simulink model "ElevatorPlant_Storage_A"  (R2015b)
(part 6 of 8)

              BUT_1=BUT_TEMP;
              FIRST_BUT=false;
            state Button_CAR_2
              en:
              BUTTON_CAR(3)=true;
              BUT_TEMP=2;
              LPC2=true;
              PUSHED=true;
              UPDATE=false;
              IN_LL=false; ET_LL=0;
            state First_but_2
              en:
              BUT_1=BUT_TEMP;
              FIRST_BUT=false;
            state Button_CAR_3
              en:
              BUTTON_CAR(4)=true;
              BUT_TEMP=3;
              LPC3=true;
              PUSHED=true;
              UPDATE=false;
              IN_LL=false; ET_LL=0;
            state First_but_3
              en:
              BUT_1=BUT_TEMP;
              FIRST_BUT=false;
            (default) -> (junction 91635)
            (junction 91635) -> Emergency.Doors.Opening0.Button_detection.BUTTON_CAR.Button_CAR_0 [order 1] : [P0]
            Emergency.Doors.Opening0.Button_detection.BUTTON_CAR.Button_CAR_0 -> (junction 91636)
            (junction 91636) -> Emergency.Doors.Opening0.Button_detection.BUTTON_CAR.First_but_0 [order 1] : [FIRST_BUT && not(RPC0)]
            Emergency.Doors.Opening0.Button_detection.BUTTON_CAR.First_but_0 -> (junction 91637)
            (junction 91635) -> (junction 91638) [order 2]
            (junction 91636) -> (junction 91639) [order 2]
            (junction 91637) -> (junction 91640)
            (junction 91639) -> (junction 91638)
            (junction 91640) -> (junction 91639)
            (junction 91638) -> (junction 91643)
            Emergency.Doors.Opening0.Button_detection.BUTTON_CAR.Button_CAR_1 -> (junction 91641)
            (junction 91641) -> Emergency.Doors.Opening0.Button_detection.BUTTON_CAR.First_but_1 [order 1] : [FIRST_BUT && not(RPC1)]
            Emergency.Doors.Opening0.Button_detection.BUTTON_CAR.First_but_1 -> (junction 91642)
            (junction 91641) -> (junction 91645) [order 2]
            (junction 91642) -> (junction 91646)
            (junction 91643) -> Emergency.Doors.Opening0.Button_detection.BUTTON_CAR.Button_CAR_1 [order 1] : [P1]
            (junction 91643) -> (junction 91644) [order 2]
            (junction 91645) -> (junction 91644)
            (junction 91646) -> (junction 91645)
            (junction 91644) -> (junction 91647)
            (junction 91647) -> Emergency.Doors.Opening0.Button_detection.BUTTON_CAR.Button_CAR_2 [order 1] : [P2]
            Emergency.Doors.Opening0.Button_detection.BUTTON_CAR.Button_CAR_2 -> (junction 91648)
            (junction 91648) -> Emergency.Doors.Opening0.Button_detection.BUTTON_CAR.First_but_2 [order 1] : [FIRST_BUT && not(RPC2)]
            Emergency.Doors.Opening0.Button_detection.BUTTON_CAR.First_but_2 -> (junction 91649)
            (junction 91647) -> (junction 91650) [order 2]
            (junction 91648) -> (junction 91651) [order 2]
            (junction 91649) -> (junction 91652)
            (junction 91651) -> (junction 91650)
            (junction 91652) -> (junction 91651)
            (junction 91650) -> (junction 91653)
            (junction 91653) -> Emergency.Doors.Opening0.Button_detection.BUTTON_CAR.Button_CAR_3 [order 1] : [P3]
            Emergency.Doors.Opening0.Button_detection.BUTTON_CAR.Button_CAR_3 -> (junction 91654)
            (junction 91654) -> Emergency.Doors.Opening0.Button_detection.BUTTON_CAR.First_but_3 [order 1] : [FIRST_BUT && not(RPC3)]
            Emergency.Doors.Opening0.Button_detection.BUTTON_CAR.First_but_3 -> (junction 91655)
            (junction 91653) -> (junction 91656) [order 2]
            (junction 91654) -> (junction 91657) [order 2]
            (junction 91655) -> (junction 91658)
            (junction 91657) -> (junction 91656)
            (junction 91658) -> (junction 91657)
          state BUTTON_UP
            state Button_UP_0
              en:
              BUTTON_UP(1)=true;
              BUT_TEMP=0;
              LPS0=true;
              PUSHED=true;
              UPDATE=false;
              IN_LL=false; ET_LL=0;
            state First_but_0
              en:
              BUT_1=BUT_TEMP;
              FIRST_BUT=false;
            state Button_UP_1
              en:
              BUTTON_UP(2)=true;
              BUT_TEMP=1;
              LPS1=true;
              PUSHED=true;
              UPDATE=false;
              IN_LL=false; ET_LL=0;
            state First_but_1
              en:
              BUT_1=BUT_TEMP;
              FIRST_BUT=false;
            state Button_UP_2
              en:
              BUTTON_UP(3)=true;
              BUT_TEMP=2;
              LPS2=true;
              PUSHED=true;
              UPDATE=false;
              IN_LL=false; ET_LL=0;
            state First_but_2
              en:
              BUT_1=BUT_TEMP;
              FIRST_BUT=false;
            (junction 91708) -> Emergency.Doors.Opening0.Button_detection.BUTTON_UP.Button_UP_0 [order 1] : [PS0]
            Emergency.Doors.Opening0.Button_detection.BUTTON_UP.Button_UP_0 -> (junction 91709)
            (junction 91709) -> Emergency.Doors.Opening0.Button_detection.BUTTON_UP.First_but_0 [order 1] : [FIRST_BUT && not(RPC0)]
            Emergency.Doors.Opening0.Button_detection.BUTTON_UP.First_but_0 -> (junction 91710)
            (default) -> (junction 91708)
            (junction 91708) -> (junction 91713) [order 2]
            (junction 91709) -> (junction 91711) [order 2]
            (junction 91710) -> (junction 91712)
            (junction 91712) -> (junction 91711)
            (junction 91711) -> (junction 91713)
            (junction 91713) -> (junction 91714)
            (junction 91714) -> Emergency.Doors.Opening0.Button_detection.BUTTON_UP.Button_UP_1 [order 1] : [PS1]
            Emergency.Doors.Opening0.Button_detection.BUTTON_UP.Button_UP_1 -> (junction 91715)
            (junction 91715) -> Emergency.Doors.Opening0.Button_detection.BUTTON_UP.First_but_1 [order 1] : [FIRST_BUT && not(RPC1)]
            Emergency.Doors.Opening0.Button_detection.BUTTON_UP.First_but_1 -> (junction 91716)
            (junction 91714) -> (junction 91717) [order 2]
            (junction 91715) -> (junction 91718) [order 2]
            (junction 91716) -> (junction 91719)
            (junction 91718) -> (junction 91717)
            (junction 91719) -> (junction 91718)
            (junction 91717) -> (junction 91721)
            Emergency.Doors.Opening0.Button_detection.BUTTON_UP.First_but_2 -> (junction 91720)
            (junction 91720) -> (junction 91725)
            (junction 91721) -> Emergency.Doors.Opening0.Button_detection.BUTTON_UP.Button_UP_2 [order 1] : [PS2]
            Emergency.Doors.Opening0.Button_detection.BUTTON_UP.Button_UP_2 -> (junction 91722)
            (junction 91722) -> Emergency.Doors.Opening0.Button_detection.BUTTON_UP.First_but_2 [order 1] : [FIRST_BUT && not(RPC2)]
            (junction 91721) -> (junction 91723) [order 2]
            (junction 91722) -> (junction 91724) [order 2]
            (junction 91724) -> (junction 91723)
            (junction 91725) -> (junction 91724)
          state Max_Min_assignment
            state Min_but
              en:
              BUTTON=MIN_BUT;
            state Max_but
              en:
              BUTTON=MAX_BUT;
            state First_but
              en:
              BUTTON=BUT_1;
            state Max_but1
              en:
              MAX_BUT=2;
            state Max_but2
              en:
              MAX_BUT=1;
            state Max_but3
              en:
              MAX_BUT=0;
            state Min_but1
              en:
              MIN_BUT=1;
            state Min_but2
              en:
              MIN_BUT=2;
            state Min_but3
              en:
              MIN_BUT=3;
            state MAX
              en:
              MAX_BUT=BUT_TEMP;
            state MIN
              en:
              MIN_BUT=BUT_TEMP;
            state Updating_button_0
              en:
              BUTTON=MAX_BUT;
            state Updating_button_1
              en:
              BUTTON=MIN_BUT;
            (junction 91763) -> Emergency.Doors.Opening0.Button_detection.Max_Min_assignment.Min_but [order 1] : [(MAX_BUT-FLOOR)>(FLOOR-MIN_BUT)]
            Emergency.Doors.Opening0.Button_detection.Max_Min_assignment.Min_but -> (junction 91764)
            (junction 91765) -> (junction 91763) [order 1] : [not(FLAG_STOP) && MOTION==2 && FLAG==3]
            (default) -> (junction 91765)
            (junction 91763) -> (junction 91766) [order 2]
            (junction 91764) -> (junction 91767)
            (junction 91765) -> (junction 91768) [order 2]
            (junction 91766) -> Emergency.Doors.Opening0.Button_detection.Max_Min_assignment.Max_but [order 1] : [(MAX_BUT-FLOOR)<(FLOOR-MIN_BUT)]
            Emergency.Doors.Opening0.Button_detection.Max_Min_assignment.Max_but -> (junction 91767)
            (junction 91766) -> Emergency.Doors.Opening0.Button_detection.Max_Min_assignment.First_but [order 2]
            (junction 91767) -> (junction 91770)
            Emergency.Doors.Opening0.Button_detection.Max_Min_assignment.First_but -> (junction 91769)
            (junction 91769) -> (junction 91768)
            (junction 91770) -> (junction 91769)
            (junction 91768) -> (junction 91771)
            (junction 91772) -> (junction 91773) [order 1] : [MOTION==0]
                | {MOTION=1;
                | UPDATE=true;}
            (junction 91773) -> Emergency.Doors.Opening0.Button_detection.Max_Min_assignment.Max_but1 [order 1] : [BUTTON_UP(2)]
            Emergency.Doors.Opening0.Button_detection.Max_Min_assignment.Max_but1 -> (junction 91774)
            (junction 91771) -> (junction 91772) [order 1] : [BUTTON==FLOOR && EXTEND]
                | {EXTEND=false;}
            (junction 91771) -> (junction 91785) [order 2]
            (junction 91772) -> (junction 91777) [order 2]
            (junction 91773) -> (junction 91775) [order 2]
            (junction 91774) -> (junction 91776)
            (junction 91775) -> Emergency.Doors.Opening0.Button_detection.Max_Min_assignment.Max_but2 [order 1] : [BUTTON_UP(1)]
            Emergency.Doors.Opening0.Button_detection.Max_Min_assignment.Max_but2 -> (junction 91776)
            (junction 91775) -> Emergency.Doors.Opening0.Button_detection.Max_Min_assignment.Max_but3 [order 2]
            (junction 91776) -> (junction 91779)
            Emergency.Doors.Opening0.Button_detection.Max_Min_assignment.Max_but3 -> (junction 91778)
            (junction 91778) -> (junction 91777)
            (junction 91779) -> (junction 91778)
            (junction 91777) -> (junction 91780)
            (junction 91780) -> (junction 91781) [order 1] : [MOTION==1]
                | {MOTION=0;
                | UPDATE=true;}
            (junction 91781) -> Emergency.Doors.Opening0.Button_detection.Max_Min_assignment.Min_but1 [order 1] : [BUTTON_DOWN(1)]
            Emergency.Doors.Opening0.Button_detection.Max_Min_assignment.Min_but1 -> (junction 91782)
            (junction 91780) -> (junction 91786) [order 2]
            (junction 91781) -> (junction 91783) [order 2]
            (junction 91782) -> (junction 91784)
            (junction 91783) -> Emergency.Doors.Opening0.Button_detection.Max_Min_assignment.Min_but2 [order 1] : [BUTTON_DOWN(2)]
            Emergency.Doors.Opening0.Button_detection.Max_Min_assignment.Min_but2 -> (junction 91784)
            (junction 91783) -> Emergency.Doors.Opening0.Button_detection.Max_Min_assignment.Min_but3 [order 2]
            (junction 91784) -> (junction 91788)
            Emergency.Doors.Opening0.Button_detection.Max_Min_assignment.Min_but3 -> (junction 91787)
            (junction 91786) -> (junction 91785)
            (junction 91787) -> (junction 91786)
            (junction 91788) -> (junction 91787)
            (junction 91785) -> (junction 91790)
            Emergency.Doors.Opening0.Button_detection.Max_Min_assignment.MAX -> (junction 91789)
            (junction 91790) -> (junction 91791) [order 1] : [PUSHED]
            (junction 91791) -> (junction 91792) [order 1] : [not(BUT_TEMP==FLOOR) || not(MOTION==2)]
            (junction 91792) -> Emergency.Doors.Opening0.Button_detection.Max_Min_assignment.MAX [order 1] : [MAX_BUT<BUT_TEMP && not(UPDATE)]
            (junction 91789) -> (junction 91794)
            (junction 91790) -> (junction 91804) [order 2]
            (junction 91791) -> (junction 91797) [order 2]
            (junction 91792) -> (junction 91793) [order 2]
            (junction 91794) -> (junction 91793)
            (junction 91793) -> (junction 91795)
            (junction 91795) -> Emergency.Doors.Opening0.Button_detection.Max_Min_assignment.MIN [order 1] : [MIN_BUT>BUT_TEMP && not(UPDATE)]
            Emergency.Doors.Opening0.Button_detection.Max_Min_assignment.MIN -> (junction 91796)
            (junction 91795) -> (junction 91798) [order 2]
            (junction 91796) -> (junction 91799)
            (junction 91798) -> (junction 91797)
            (junction 91799) -> (junction 91798)
            (junction 91797) -> (junction 91800)
            (junction 91800) -> Emergency.Doors.Opening0.Button_detection.Max_Min_assignment.Updating_button_0 [order 1] : [MOTION==0]
            Emergency.Doors.Opening0.Button_detection.Max_Min_assignment.Updating_button_0 -> (junction 91801)
            (junction 91800) -> (junction 91802) [order 2]
            (junction 91801) -> (junction 91803)
            (junction 91802) -> Emergency.Doors.Opening0.Button_detection.Max_Min_assignment.Updating_button_1 [order 1] : [MOTION==1]
            Emergency.Doors.Opening0.Button_detection.Max_Min_assignment.Updating_button_1 -> (junction 91803)
            (junction 91802) -> (junction 91805) [order 2]
            (junction 91803) -> (junction 91806)
            (junction 91805) -> (junction 91804)
            (junction 91806) -> (junction 91805)
          state GoTo_PositionControl
            en:
            BUTTON=BUT_TEMP;
            FLAG=2;
          state Emergency
            en:
            FLAG_EMG=true;
            FLAG=4;
          state Timer_EME
            state Set_tmr
              en:
              Q_EME=true;
            state Counting
              en:
              ET_EME= ET_EME + 1;
              Q_EME=false;
            state Set
              en:
              IN_EME=true;
              PT_EME=3;
            (junction 91896) -> Emergency.Doors.Opening0.Button_detection.Timer_EME.Set_tmr [order 1] : [ET_EME==PT_EME]
            Emergency.Doors.Opening0.Button_detection.Timer_EME.Set_tmr -> (junction 91897)
            Emergency.Doors.Opening0.Button_detection.Timer_EME.Counting -> (junction 91896)
            (junction 91896) -> (junction 91897) [order 2]
            (default) -> Emergency.Doors.Opening0.Button_detection.Timer_EME.Set
            Emergency.Doors.Opening0.Button_detection.Timer_EME.Set -> (junction 91898)
            (junction 91898) -> Emergency.Doors.Opening0.Button_detection.Timer_EME.Counting [order 1] : [ET_EME<PT_EME]
            (junction 91898) -> (junction 91897) [order 2]
          state Not_Emergency
            en:
            IN_EME=false;
            ET_EME=0;
          state SwitchingOFF_LEDs
            en:
            LPD3=false;
            LPD2=false;
            LPS2=false;
            LPD1=false;
            LPS1=false;
            LPS0=false;
          (default) -> (junction 91497)
          (junction 91497) -> (junction 91498) [order 1] : [FLAG==1 && not(PUSHED)]
              | {BUTTON=FLOOR;
              | BUT_TEMP=BUTTON;
              | BUT_1=FLOOR;}
          (junction 91498) -> Emergency.Doors.Opening0.Button_detection.Timer_LL [order 1] : [not(FLAG_STOP)]
          Emergency.Doors.Opening0.Button_detection.Timer_LL -> Emergency.Doors.Opening0.Button_detection.Save_energy
          Emergency.Doors.Opening0.Button_detection.Save_energy -> (junction 91499)
          (junction 91497) -> (junction 91500) [order 2]
          (junction 91498) -> (junction 91501) [order 2]
          (junction 91499) -> (junction 91502)
          (junction 91501) -> (junction 91500)
          (junction 91502) -> (junction 91501)
          (junction 91500) -> Emergency.Doors.Opening0.Button_detection.BUTTON_CAR
          Emergency.Doors.Opening0.Button_detection.BUTTON_UP -> Emergency.Doors.Opening0.Button_detection.BUTTON_DOWN
          Emergency.Doors.Opening0.Button_detection.BUTTON_DOWN -> Emergency.Doors.Opening0.Button_detection.Max_Min_assignment
          Emergency.Doors.Opening0.Button_detection.Max_Min_assignment -> (junction 91503)
          Emergency.Doors.Opening0.Button_detection.BUTTON_CAR -> Emergency.Doors.Opening0.Button_detection.BUTTON_UP
          (junction 91503) -> (junction 91505)
          (junction 91505) -> (junction 91504)
          (junction 91504) -> (junction 91506)
          (junction 91506) -> (junction 91507) [order 1] : [FLAG==1]
          (junction 91507) -> Emergency.Doors.Opening0.Button_detection.GoTo_PositionControl [order 1] : [PUSHED]
          Emergency.Doors.Opening0.Button_detection.GoTo_PositionControl -> (junction 91508)
          (junction 91506) -> (junction 91518) [order 2]
          (junction 91507) -> (junction 91509) [order 2]
          (junction 91508) -> (junction 91510)
          (junction 91510) -> (junction 91509)
          (junction 91509) -> (junction 91512)
          Emergency.Doors.Opening0.Button_detection.Emergency -> (junction 91511)
          (junction 91512) -> Emergency.Doors.Opening0.Button_detection.Timer_EME [order 1] : [STOP]
              | {IN_LL=false; ET_LL=0;FLAG=1;}
          Emergency.Doors.Opening0.Button_detection.Timer_EME -> (junction 91513)
          (junction 91513) -> Emergency.Doors.Opening0.Button_detection.Emergency [order 1] : [Q_EME]
          (junction 91511) -> (junction 91515)
          (junction 91512) -> Emergency.Doors.Opening0.Button_detection.Not_Emergency [order 2]
          (junction 91513) -> (junction 91514) [order 2]
          (junction 91515) -> (junction 91514)
          (junction 91514) -> (junction 91517)
          Emergency.Doors.Opening0.Button_detection.Not_Emergency -> (junction 91517)
          Emergency.Doors.Opening0.Button_detection.SwitchingOFF_LEDs -> (junction 91516)
          (junction 91517) -> Emergency.Doors.Opening0.Button_detection.SwitchingOFF_LEDs [order 1] : [FLAG_STOP && FLAG==2]
          (junction 91516) -> (junction 91520)
          (junction 91517) -> (junction 91519) [order 2]
          (junction 91519) -> (junction 91518)
          (junction 91520) -> (junction 91519)
        state Button_detection1
          state Save_energy
            en:
            LL=not(Q_LL);
          state Timer_LL
            state Set_tmr
              en:
              Q_LL=true;
            state Counting
              en:
              ET_LL= ET_LL + 1;
              Q_LL=false;
            state Set
              en:
              IN_LL=true;
              PT_LL=10;
            (junction 91981) -> Emergency.Doors.Opening0.Button_detection1.Timer_LL.Set_tmr [order 1] : [ET_LL==PT_LL]
            Emergency.Doors.Opening0.Button_detection1.Timer_LL.Set_tmr -> (junction 91982)
            Emergency.Doors.Opening0.Button_detection1.Timer_LL.Counting -> (junction 91981)
            (junction 91981) -> (junction 91982) [order 2]
            (default) -> Emergency.Doors.Opening0.Button_detection1.Timer_LL.Set
            Emergency.Doors.Opening0.Button_detection1.Timer_LL.Set -> (junction 91983)
            (junction 91983) -> Emergency.Doors.Opening0.Button_detection1.Timer_LL.Counting [order 1] : [ET_LL<PT_LL]
            (junction 91983) -> (junction 91982) [order 2]
          state BUTTON_DOWN
            state Button_DOWN_1
              en:
              BUTTON_DOWN(2)=true;
              BUT_TEMP=1;
              LPD1=true;
              PUSHED=true;
              UPDATE=false;
              IN_LL=false; ET_LL=0;
            state First_but_1
              en:
              BUT_1=BUT_TEMP;
              FIRST_BUT=false;
            state Button_DOWN_2
              en:
              BUTTON_DOWN(3)=true;
              BUT_TEMP=2;
              LPD2=true;
              PUSHED=true;
              UPDATE=false;
              IN_LL=false; ET_LL=0;
            state First_but_2
              en:
              BUT_1=BUT_TEMP;
              FIRST_BUT=false;
            state Button_DOWN_3
              en:
              BUTTON_DOWN(4)=true;
              BUT_TEMP=3;
              LPD3=true;
              PUSHED=true;
              UPDATE=false;
              IN_LL=false; ET_LL=0;
            state First_but_3
              en:
              BUT_1=BUT_TEMP;
              FIRST_BUT=false;
            (default) -> (junction 91996)
            (junction 91996) -> Emergency.Doors.Opening0.Button_detection1.BUTTON_DOWN.Button_DOWN_1 [order 1] : [PD1]
            Emergency.Doors.Opening0.Button_detection1.BUTTON_DOWN.Button_DOWN_1 -> (junction 91997)
            (junction 91997) -> Emergency.Doors.Opening0.Button_detection1.BUTTON_DOWN.First_but_1 [order 1] : [FIRST_BUT && not(RPC1)]
            Emergency.Doors.Opening0.Button_detection1.BUTTON_DOWN.First_but_1 -> (junction 91998)
            (junction 91996) -> (junction 91999) [order 2]
            (junction 91997) -> (junction 92000) [order 2]
            (junction 91998) -> (junction 92001)
            (junction 92000) -> (junction 91999)
            (junction 92001) -> (junction 92000)
            (junction 91999) -> (junction 92002)
            (junction 92002) -> Emergency.Doors.Opening0.Button_detection1.BUTTON_DOWN.Button_DOWN_2 [order 1] : [PD2]
            Emergency.Doors.Opening0.Button_detection1.BUTTON_DOWN.Button_DOWN_2 -> (junction 92003)
            (junction 92003) -> Emergency.Doors.Opening0.Button_detection1.BUTTON_DOWN.First_but_2 [order 1] : [FIRST_BUT && not(RPC2)]
            Emergency.Doors.Opening0.Button_detection1.BUTTON_DOWN.First_but_2 -> (junction 92004)
            (junction 92002) -> (junction 92005) [order 2]
            (junction 92003) -> (junction 92006) [order 2]
            (junction 92004) -> (junction 92007)
            (junction 92006) -> (junction 92005)
            (junction 92007) -> (junction 92006)
            (junction 92005) -> (junction 92008)
            (junction 92008) -> Emergency.Doors.Opening0.Button_detection1.BUTTON_DOWN.Button_DOWN_3 [order 1] : [PD3]
            Emergency.Doors.Opening0.Button_detection1.BUTTON_DOWN.Button_DOWN_3 -> (junction 92009)
            (junction 92009) -> Emergency.Doors.Opening0.Button_detection1.BUTTON_DOWN.First_but_3 [order 1] : [FIRST_BUT && not(RPC3)]
            Emergency.Doors.Opening0.Button_detection1.BUTTON_DOWN.First_but_3 -> (junction 92010)
            (junction 92008) -> (junction 92011) [order 2]
            (junction 92009) -> (junction 92012) [order 2]
            (junction 92010) -> (junction 92013)
            (junction 92012) -> (junction 92011)
            (junction 92013) -> (junction 92012)
          state BUTTON_CAR
            state Button_CAR_0
              en:
              BUTTON_CAR(1)=true;
              BUT_TEMP=0;
              LPC0=true;
              PUSHED=true;
              UPDATE=false;
              IN_LL=false; ET_LL=0;
            state First_but_0
              en:
              BUT_1=BUT_TEMP;
              FIRST_BUT=false;
            state Button_CAR_1
              en:
              BUTTON_CAR(2)=true;
              BUT_TEMP=1;
              LPC1=true;
              PUSHED=true;
              UPDATE=false;
              IN_LL=false; ET_LL=0;
            state First_but_1
              en:
              BUT_1=BUT_TEMP;
              FIRST_BUT=false;
            state Button_CAR_2
              en:
              BUTTON_CAR(3)=true;
              BUT_TEMP=2;
              LPC2=true;
              PUSHED=true;
              UPDATE=false;
              IN_LL=false; ET_LL=0;
            state First_but_2
              en:
              BUT_1=BUT_TEMP;
              FIRST_BUT=false;
            state Button_CAR_3
              en:
              BUTTON_CAR(4)=true;
              BUT_TEMP=3;
              LPC3=true;
              PUSHED=true;
              UPDATE=false;
              IN_LL=false; ET_LL=0;
            state First_but_3
              en:
              BUT_1=BUT_TEMP;
              FIRST_BUT=false;
            (default) -> (junction 92051)
            (junction 92051) -> Emergency.Doors.Opening0.Button_detection1.BUTTON_CAR.Button_CAR_0 [order 1] : [P0]
            Emergency.Doors.Opening0.Button_detection1.BUTTON_CAR.Button_CAR_0 -> (junction 92052)
            (junction 92052) -> Emergency.Doors.Opening0.Button_detection1.BUTTON_CAR.First_but_0 [order 1] : [FIRST_BUT && not(RPC0)]
            Emergency.Doors.Opening0.Button_detection1.BUTTON_CAR.First_but_0 -> (junction 92053)
            (junction 92051) -> (junction 92054) [order 2]
            (junction 92052) -> (junction 92055) [order 2]
            (junction 92053) -> (junction 92056)
            (junction 92055) -> (junction 92054)
            (junction 92056) -> (junction 92055)
            (junction 92054) -> (junction 92059)
            Emergency.Doors.Opening0.Button_detection1.BUTTON_CAR.Button_CAR_1 -> (junction 92057)
            (junction 92057) -> Emergency.Doors.Opening0.Button_detection1.BUTTON_CAR.First_but_1 [order 1] : [FIRST_BUT && not(RPC1)]
            Emergency.Doors.Opening0.Button_detection1.BUTTON_CAR.First_but_1 -> (junction 92058)
            (junction 92057) -> (junction 92061) [order 2]
            (junction 92058) -> (junction 92062)
            (junction 92059) -> Emergency.Doors.Opening0.Button_detection1.BUTTON_CAR.Button_CAR_1 [order 1] : [P1]
            (junction 92059) -> (junction 92060) [order 2]
            (junction 92061) -> (junction 92060)
            (junction 92062) -> (junction 92061)
            (junction 92060) -> (junction 92063)
            (junction 92063) -> Emergency.Doors.Opening0.Button_detection1.BUTTON_CAR.Button_CAR_2 [order 1] : [P2]
            Emergency.Doors.Opening0.Button_detection1.BUTTON_CAR.Button_CAR_2 -> (junction 92064)
            (junction 92064) -> Emergency.Doors.Opening0.Button_detection1.BUTTON_CAR.First_but_2 [order 1] : [FIRST_BUT && not(RPC2)]
            Emergency.Doors.Opening0.Button_detection1.BUTTON_CAR.First_but_2 -> (junction 92065)
            (junction 92063) -> (junction 92066) [order 2]
            (junction 92064) -> (junction 92067) [order 2]
            (junction 92065) -> (junction 92068)
            (junction 92067) -> (junction 92066)
            (junction 92068) -> (junction 92067)
            (junction 92066) -> (junction 92069)
            (junction 92069) -> Emergency.Doors.Opening0.Button_detection1.BUTTON_CAR.Button_CAR_3 [order 1] : [P3]
            Emergency.Doors.Opening0.Button_detection1.BUTTON_CAR.Button_CAR_3 -> (junction 92070)
            (junction 92070) -> Emergency.Doors.Opening0.Button_detection1.BUTTON_CAR.First_but_3 [order 1] : [FIRST_BUT && not(RPC3)]
            Emergency.Doors.Opening0.Button_detection1.BUTTON_CAR.First_but_3 -> (junction 92071)
            (junction 92069) -> (junction 92072) [order 2]
            (junction 92070) -> (junction 92073) [order 2]
            (junction 92071) -> (junction 92074)
            (junction 92073) -> (junction 92072)
            (junction 92074) -> (junction 92073)
          state BUTTON_UP
            state Button_UP_0
              en:
              BUTTON_UP(1)=true;
              BUT_TEMP=0;
              LPS0=true;
              PUSHED=true;
              UPDATE=false;
              IN_LL=false; ET_LL=0;
            state First_but_0
              en:
              BUT_1=BUT_TEMP;
              FIRST_BUT=false;
            state Button_UP_1
              en:
              BUTTON_UP(2)=true;
              BUT_TEMP=1;
              LPS1=true;
              PUSHED=true;
              UPDATE=false;
              IN_LL=false; ET_LL=0;
            state First_but_1
              en:
              BUT_1=BUT_TEMP;
              FIRST_BUT=false;
            state Button_UP_2
              en:
              BUTTON_UP(3)=true;
              BUT_TEMP=2;
              LPS2=true;
              PUSHED=true;
              UPDATE=false;
              IN_LL=false; ET_LL=0;
            state First_but_2
              en:
              BUT_1=BUT_TEMP;
              FIRST_BUT=false;
            (junction 92124) -> Emergency.Doors.Opening0.Button_detection1.BUTTON_UP.Button_UP_0 [order 1] : [PS0]
            Emergency.Doors.Opening0.Button_detection1.BUTTON_UP.Button_UP_0 -> (junction 92125)
            (junction 92125) -> Emergency.Doors.Opening0.Button_detection1.BUTTON_UP.First_but_0 [order 1] : [FIRST_BUT && not(RPC0)]
            Emergency.Doors.Opening0.Button_detection1.BUTTON_UP.First_but_0 -> (junction 92126)
            (default) -> (junction 92124)
            (junction 92124) -> (junction 92129) [order 2]
            (junction 92125) -> (junction 92127) [order 2]
            (junction 92126) -> (junction 92128)
            (junction 92128) -> (junction 92127)
            (junction 92127) -> (junction 92129)
            (junction 92129) -> (junction 92130)
            (junction 92130) -> Emergency.Doors.Opening0.Button_detection1.BUTTON_UP.Button_UP_1 [order 1] : [PS1]
            Emergency.Doors.Opening0.Button_detection1.BUTTON_UP.Button_UP_1 -> (junction 92131)
            (junction 92131) -> Emergency.Doors.Opening0.Button_detection1.BUTTON_UP.First_but_1 [order 1] : [FIRST_BUT && not(RPC1)]
            Emergency.Doors.Opening0.Button_detection1.BUTTON_UP.First_but_1 -> (junction 92132)
            (junction 92130) -> (junction 92133) [order 2]
            (junction 92131) -> (junction 92134) [order 2]
            (junction 92132) -> (junction 92135)
            (junction 92134) -> (junction 92133)
            (junction 92135) -> (junction 92134)
            (junction 92133) -> (junction 92137)
            Emergency.Doors.Opening0.Button_detection1.BUTTON_UP.First_but_2 -> (junction 92136)
            (junction 92136) -> (junction 92141)
            (junction 92137) -> Emergency.Doors.Opening0.Button_detection1.BUTTON_UP.Button_UP_2 [order 1] : [PS2]
            Emergency.Doors.Opening0.Button_detection1.BUTTON_UP.Button_UP_2 -> (junction 92138)
            (junction 92138) -> Emergency.Doors.Opening0.Button_detection1.BUTTON_UP.First_but_2 [order 1] : [FIRST_BUT && not(RPC2)]
            (junction 92137) -> (junction 92139) [order 2]
            (junction 92138) -> (junction 92140) [order 2]
            (junction 92140) -> (junction 92139)
            (junction 92141) -> (junction 92140)
          state Max_Min_assignment
            state Min_but
              en:
              BUTTON=MIN_BUT;
            state Max_but
              en:
              BUTTON=MAX_BUT;
            state First_but
              en:
              BUTTON=BUT_1;
            state Max_but1
              en:
              MAX_BUT=2;
            state Max_but2
              en:
              MAX_BUT=1;
            state Max_but3
              en:
              MAX_BUT=0;
            state Min_but1
              en:
              MIN_BUT=1;
            state Min_but2
              en:
              MIN_BUT=2;
            state Min_but3
              en:
              MIN_BUT=3;
            state MAX
              en:
              MAX_BUT=BUT_TEMP;
            state MIN
              en:
              MIN_BUT=BUT_TEMP;
            state Updating_button_0
              en:
              BUTTON=MAX_BUT;
            state Updating_button_1
              en:
              BUTTON=MIN_BUT;
            (junction 92179) -> Emergency.Doors.Opening0.Button_detection1.Max_Min_assignment.Min_but [order 1] : [(MAX_BUT-FLOOR)>(FLOOR-MIN_BUT)]
            Emergency.Doors.Opening0.Button_detection1.Max_Min_assignment.Min_but -> (junction 92180)
            (junction 92181) -> (junction 92179) [order 1] : [not(FLAG_STOP) && MOTION==2 && FLAG==3]
            (default) -> (junction 92181)
            (junction 92179) -> (junction 92182) [order 2]
            (junction 92180) -> (junction 92183)
            (junction 92181) -> (junction 92184) [order 2]
            (junction 92182) -> Emergency.Doors.Opening0.Button_detection1.Max_Min_assignment.Max_but [order 1] : [(MAX_BUT-FLOOR)<(FLOOR-MIN_BUT)]
            Emergency.Doors.Opening0.Button_detection1.Max_Min_assignment.Max_but -> (junction 92183)
            (junction 92182) -> Emergency.Doors.Opening0.Button_detection1.Max_Min_assignment.First_but [order 2]
            (junction 92183) -> (junction 92186)
            Emergency.Doors.Opening0.Button_detection1.Max_Min_assignment.First_but -> (junction 92185)
            (junction 92185) -> (junction 92184)
            (junction 92186) -> (junction 92185)
            (junction 92184) -> (junction 92187)
            (junction 92188) -> (junction 92189) [order 1] : [MOTION==0]
                | {MOTION=1;
                | UPDATE=true;}
            (junction 92189) -> Emergency.Doors.Opening0.Button_detection1.Max_Min_assignment.Max_but1 [order 1] : [BUTTON_UP(2)]
            Emergency.Doors.Opening0.Button_detection1.Max_Min_assignment.Max_but1 -> (junction 92190)
            (junction 92187) -> (junction 92188) [order 1] : [BUTTON==FLOOR && EXTEND]
                | {EXTEND=false;}
            (junction 92187) -> (junction 92201) [order 2]
            (junction 92188) -> (junction 92193) [order 2]
            (junction 92189) -> (junction 92191) [order 2]
            (junction 92190) -> (junction 92192)
            (junction 92191) -> Emergency.Doors.Opening0.Button_detection1.Max_Min_assignment.Max_but2 [order 1] : [BUTTON_UP(1)]
            Emergency.Doors.Opening0.Button_detection1.Max_Min_assignment.Max_but2 -> (junction 92192)
            (junction 92191) -> Emergency.Doors.Opening0.Button_detection1.Max_Min_assignment.Max_but3 [order 2]
            (junction 92192) -> (junction 92195)
            Emergency.Doors.Opening0.Button_detection1.Max_Min_assignment.Max_but3 -> (junction 92194)
            (junction 92194) -> (junction 92193)
            (junction 92195) -> (junction 92194)
            (junction 92193) -> (junction 92196)
            (junction 92196) -> (junction 92197) [order 1] : [MOTION==1]
                | {MOTION=0;
                | UPDATE=true;}
            (junction 92197) -> Emergency.Doors.Opening0.Button_detection1.Max_Min_assignment.Min_but1 [order 1] : [BUTTON_DOWN(1)]
            Emergency.Doors.Opening0.Button_detection1.Max_Min_assignment.Min_but1 -> (junction 92198)
            (junction 92196) -> (junction 92202) [order 2]
            (junction 92197) -> (junction 92199) [order 2]
            (junction 92198) -> (junction 92200)
            (junction 92199) -> Emergency.Doors.Opening0.Button_detection1.Max_Min_assignment.Min_but2 [order 1] : [BUTTON_DOWN(2)]
            Emergency.Doors.Opening0.Button_detection1.Max_Min_assignment.Min_but2 -> (junction 92200)
            (junction 92199) -> Emergency.Doors.Opening0.Button_detection1.Max_Min_assignment.Min_but3 [order 2]
            (junction 92200) -> (junction 92204)
            Emergency.Doors.Opening0.Button_detection1.Max_Min_assignment.Min_but3 -> (junction 92203)
            (junction 92202) -> (junction 92201)
            (junction 92203) -> (junction 92202)
            (junction 92204) -> (junction 92203)
            (junction 92201) -> (junction 92206)
            Emergency.Doors.Opening0.Button_detection1.Max_Min_assignment.MAX -> (junction 92205)
            (junction 92206) -> (junction 92207) [order 1] : [PUSHED]
            (junction 92207) -> (junction 92208) [order 1] : [not(BUT_TEMP==FLOOR) || not(MOTION==2)]
            (junction 92208) -> Emergency.Doors.Opening0.Button_detection1.Max_Min_assignment.MAX [order 1] : [MAX_BUT<BUT_TEMP && not(UPDATE)]
            (junction 92205) -> (junction 92210)
            (junction 92206) -> (junction 92220) [order 2]
            (junction 92207) -> (junction 92213) [order 2]
            (junction 92208) -> (junction 92209) [order 2]
            (junction 92210) -> (junction 92209)
            (junction 92209) -> (junction 92211)
            (junction 92211) -> Emergency.Doors.Opening0.Button_detection1.Max_Min_assignment.MIN [order 1] : [MIN_BUT>BUT_TEMP && not(UPDATE)]
            Emergency.Doors.Opening0.Button_detection1.Max_Min_assignment.MIN -> (junction 92212)
            (junction 92211) -> (junction 92214) [order 2]
            (junction 92212) -> (junction 92215)
            (junction 92214) -> (junction 92213)
            (junction 92215) -> (junction 92214)
            (junction 92213) -> (junction 92216)
            (junction 92216) -> Emergency.Doors.Opening0.Button_detection1.Max_Min_assignment.Updating_button_0 [order 1] : [MOTION==0]
            Emergency.Doors.Opening0.Button_detection1.Max_Min_assignment.Updating_button_0 -> (junction 92217)
            (junction 92216) -> (junction 92218) [order 2]
            (junction 92217) -> (junction 92219)
            (junction 92218) -> Emergency.Doors.Opening0.Button_detection1.Max_Min_assignment.Updating_button_1 [order 1] : [MOTION==1]
            Emergency.Doors.Opening0.Button_detection1.Max_Min_assignment.Updating_button_1 -> (junction 92219)
            (junction 92218) -> (junction 92221) [order 2]
            (junction 92219) -> (junction 92222)
            (junction 92221) -> (junction 92220)
            (junction 92222) -> (junction 92221)
          state GoTo_PositionControl
            en:
            BUTTON=BUT_TEMP;
            FLAG=2;
          state Emergency
            en:
            FLAG_EMG=true;
            FLAG=4;
          state Timer_EME
            state Set_tmr
              en:
              Q_EME=true;
            state Counting
              en:
              ET_EME= ET_EME + 1;
              Q_EME=false;
            state Set
              en:
              IN_EME=true;
              PT_EME=3;
            (junction 92312) -> Emergency.Doors.Opening0.Button_detection1.Timer_EME.Set_tmr [order 1] : [ET_EME==PT_EME]
            Emergency.Doors.Opening0.Button_detection1.Timer_EME.Set_tmr -> (junction 92313)
            Emergency.Doors.Opening0.Button_detection1.Timer_EME.Counting -> (junction 92312)
            (junction 92312) -> (junction 92313) [order 2]
            (default) -> Emergency.Doors.Opening0.Button_detection1.Timer_EME.Set
            Emergency.Doors.Opening0.Button_detection1.Timer_EME.Set -> (junction 92314)
            (junction 92314) -> Emergency.Doors.Opening0.Button_detection1.Timer_EME.Counting [order 1] : [ET_EME<PT_EME]
            (junction 92314) -> (junction 92313) [order 2]
          state Not_Emergency
            en:
            IN_EME=false;
            ET_EME=0;
          state SwitchingOFF_LEDs
            en:
            LPD3=false;
            LPD2=false;
            LPS2=false;
            LPD1=false;
            LPS1=false;
            LPS0=false;
          (default) -> (junction 91913)
          (junction 91913) -> (junction 91914) [order 1] : [FLAG==1 && not(PUSHED)]
              | {BUTTON=FLOOR;
              | BUT_TEMP=BUTTON;
              | BUT_1=FLOOR;}
          (junction 91914) -> Emergency.Doors.Opening0.Button_detection1.Timer_LL [order 1] : [not(FLAG_STOP)]
          Emergency.Doors.Opening0.Button_detection1.Save_energy -> (junction 91915)
          Emergency.Doors.Opening0.Button_detection1.Timer_LL -> Emergency.Doors.Opening0.Button_detection1.Save_energy
          (junction 91914) -> (junction 91917) [order 2]
          (junction 91913) -> (junction 91916) [order 2]
          (junction 91915) -> (junction 91918)
          (junction 91917) -> (junction 91916)
          (junction 91918) -> (junction 91917)
          (junction 91916) -> Emergency.Doors.Opening0.Button_detection1.BUTTON_CAR
          Emergency.Doors.Opening0.Button_detection1.BUTTON_UP -> Emergency.Doors.Opening0.Button_detection1.BUTTON_DOWN
          Emergency.Doors.Opening0.Button_detection1.BUTTON_DOWN -> Emergency.Doors.Opening0.Button_detection1.Max_Min_assignment
          Emergency.Doors.Opening0.Button_detection1.Max_Min_assignment -> (junction 91919)
          Emergency.Doors.Opening0.Button_detection1.BUTTON_CAR -> Emergency.Doors.Opening0.Button_detection1.BUTTON_UP
          (junction 91919) -> (junction 91921)
          (junction 91921) -> (junction 91920)
          (junction 91920) -> (junction 91923)
          Emergency.Doors.Opening0.Button_detection1.GoTo_PositionControl -> (junction 91922)
          (junction 91923) -> (junction 91924) [order 1] : [FLAG==1]
          (junction 91924) -> Emergency.Doors.Opening0.Button_detection1.GoTo_PositionControl [order 1] : [PUSHED]
          (junction 91922) -> (junction 91926)
          (junction 91923) -> (junction 91934) [order 2]
          (junction 91924) -> (junction 91925) [order 2]
          (junction 91926) -> (junction 91925)
          (junction 91925) -> (junction 91928)
          Emergency.Doors.Opening0.Button_detection1.Emergency -> (junction 91927)
          (junction 91928) -> Emergency.Doors.Opening0.Button_detection1.Timer_EME [order 1] : [STOP]
              | {IN_LL=false; ET_LL=0;FLAG=1;}
          Emergency.Doors.Opening0.Button_detection1.Timer_EME -> (junction 91929)
          (junction 91929) -> Emergency.Doors.Opening0.Button_detection1.Emergency [order 1] : [Q_EME]
          (junction 91927) -> (junction 91931)
          (junction 91928) -> Emergency.Doors.Opening0.Button_detection1.Not_Emergency [order 2]
          (junction 91929) -> (junction 91930) [order 2]
          (junction 91931) -> (junction 91930)
          (junction 91930) -> (junction 91933)
          Emergency.Doors.Opening0.Button_detection1.Not_Emergency -> (junction 91933)
          Emergency.Doors.Opening0.Button_detection1.SwitchingOFF_LEDs -> (junction 91932)
          (junction 91933) -> Emergency.Doors.Opening0.Button_detection1.SwitchingOFF_LEDs [order 1] : [FLAG_STOP && FLAG==2]
          (junction 91932) -> (junction 91936)
          (junction 91933) -> (junction 91935) [order 2]
          (junction 91935) -> (junction 91934)
          (junction 91936) -> (junction 91935)
        state Opening1
          en:AP0=true;
        state Reset
          state Reset_0
            en:
            LPS0=false;
            BUTTON_CAR(1)=false;
            BUTTON_UP(1)=false;
          state Reset_1
            en:
            LPS1=false;
            LPD1=false;
            BUTTON_CAR(2)=false;
            BUTTON_UP(2)=false;
            BUTTON_DOWN(2)=false;
          state Reset_2
            en:
            LPS2=false;
            LPD2=false;
            BUTTON_CAR(3)=false;
            BUTTON_UP(3)=false;
            BUTTON_DOWN(3)=false;
          state Reset_3
            en:
            LPD3=false;
            BUTTON_CAR(4)=false;
            BUTTON_DOWN(4)=false;
          (default) -> (junction 92330)
          (junction 92330) -> Emergency.Doors.Opening0.Reset.Reset_0 [order 1] : [FLOOR==0]
          Emergency.Doors.Opening0.Reset.Reset_0 -> (junction 92331)
          (junction 92330) -> (junction 92332) [order 2]
          (junction 92331) -> (junction 92333)
          (junction 92332) -> Emergency.Doors.Opening0.Reset.Reset_1 [order 1] : [FLOOR==1]
          Emergency.Doors.Opening0.Reset.Reset_1 -> (junction 92333)
          (junction 92332) -> (junction 92334) [order 2]
          (junction 92333) -> (junction 92335)
          (junction 92334) -> Emergency.Doors.Opening0.Reset.Reset_2 [order 1] : [FLOOR==2]
          Emergency.Doors.Opening0.Reset.Reset_2 -> (junction 92335)
          (junction 92334) -> (junction 92336) [order 2]
          (junction 92335) -> (junction 92337)
          (junction 92336) -> Emergency.Doors.Opening0.Reset.Reset_3 [order 1] : [FLOOR==3]
          Emergency.Doors.Opening0.Reset.Reset_3 -> (junction 92337)
          (junction 92336) -> (junction 92338) [order 2]
          (junction 92337) -> (junction 92339)
          (junction 92339) -> (junction 92338)
        state Stop_Opening1
          en: AP0=false;
          FLAG_OD=true;
          IN_cl=false;
          ET_cl=0;
        (junction 91327) -> (junction 91328)
        (junction 91328) -> (junction 91329) [order 1] : [not(OBS) ]
        (junction 91329) -> (junction 91330) [order 2]
        (junction 91330) -> Emergency.Doors.Opening0.Timer_open
        Emergency.Doors.Opening0.Timer_open -> (junction 91331)
        (junction 91331) -> Emergency.Doors.Opening0.Opening [order 1] : [not(PA0)]
        (default) -> Emergency.Doors.Opening0.People_IN
        (junction 91328) -> (junction 91332) [order 2]
        (junction 91329) -> Emergency.Doors.Opening0.Button_detection [order 1] : [not(FLAG==4)]
        (junction 91334) -> (junction 91330)
        (junction 91336) -> (junction 91327)
        (junction 91331) -> Emergency.Doors.Opening0.Stop_Opening [order 2]
        Emergency.Doors.Opening0.People_IN -> Emergency.Doors.Opening0.People_OUT
        Emergency.Doors.Opening0.Opening -> (junction 91341)
        (junction 91332) -> (junction 91333) [order 2]
        (junction 91332) -> Emergency.Doors.Opening0.Button_detection1 [order 1] : [not(FLAG==4)]
        (junction 91333) -> (junction 91338)
        Emergency.Doors.Opening0.Button_detection -> (junction 91334)
        Emergency.Doors.Opening0.People_OUT -> (junction 91335)
        Emergency.Doors.Opening0.Button_detection1 -> (junction 91337)
        (junction 91338) -> (junction 91337)
        (junction 91335) -> (junction 91336) [order 2]
        (junction 91335) -> Emergency.Doors.Opening0.Reset [order 1] : [not(FLAG==4)]
        (junction 91337) -> (junction 91339)
        (junction 91345) -> (junction 91336)
        Emergency.Doors.Opening0.Stop_Opening -> (junction 91340)
        (junction 91339) -> Emergency.Doors.Opening0.Opening1 [order 1] : [not(PA0)]
        (junction 91339) -> Emergency.Doors.Opening0.Stop_Opening1 [order 2]
        (junction 91341) -> (junction 91340)
        (junction 91340) -> (junction 91343)
        Emergency.Doors.Opening0.Opening1 -> (junction 91342)
        Emergency.Doors.Opening0.Reset -> (junction 91344)
        Emergency.Doors.Opening0.Stop_Opening1 -> (junction 91342)
        (junction 91342) -> (junction 91343)
        (junction 91344) -> (junction 91345)
      state FLOOR_1
        en: CP1=false;
      state Opening1
        state Opening
          en:AP1=Q_op;
        state People_IN
          state Check_People_IN
            en:
            COUNTER_IN=false;
          state People_KID_IN
            en:
            WEIGHT=WEIGHT+30;
            KIDS=KIDS+1;
          state People_WOMAN_IN
            en:
            WEIGHT=WEIGHT+55;
            WOMEN=WOMEN+1;
          state People_MAN_IN
            en:
            WEIGHT=WEIGHT+75;
            MEN=MEN+1;
          state People_FATGUY_IN
            en:
            WEIGHT=WEIGHT+100;
            FATGUYS=FATGUYS+1;
          state Re_Ready_IN
            en:
            COUNTER_IN=true;
          (default) -> (junction 92420)
          (junction 92420) -> Emergency.Doors.Opening1.People_IN.Check_People_IN [order 1] : [COUNTER_IN]
          Emergency.Doors.Opening1.People_IN.Check_People_IN -> (junction 92421)
          (junction 92421) -> Emergency.Doors.Opening1.People_IN.People_KID_IN [order 1] : [KID_IN]
          Emergency.Doors.Opening1.People_IN.People_KID_IN -> (junction 92422)
          (junction 92420) -> (junction 92429) [order 2]
          (junction 92421) -> (junction 92423) [order 2]
          (junction 92422) -> (junction 92424)
          (junction 92423) -> Emergency.Doors.Opening1.People_IN.People_WOMAN_IN [order 1] : [WOMAN_IN]
          Emergency.Doors.Opening1.People_IN.People_WOMAN_IN -> (junction 92424)
          (junction 92423) -> (junction 92425) [order 2]
          (junction 92424) -> (junction 92426)
          (junction 92425) -> Emergency.Doors.Opening1.People_IN.People_MAN_IN [order 1] : [MAN_IN]
          Emergency.Doors.Opening1.People_IN.People_MAN_IN -> (junction 92426)
          (junction 92425) -> (junction 92427) [order 2]
          (junction 92426) -> (junction 92428)
          (junction 92427) -> Emergency.Doors.Opening1.People_IN.People_FATGUY_IN [order 1] : [FATGUY_IN]
          Emergency.Doors.Opening1.People_IN.People_FATGUY_IN -> (junction 92428)
          (junction 92427) -> (junction 92430) [order 2]
          (junction 92428) -> (junction 92431)
          (junction 92430) -> (junction 92429)
          (junction 92431) -> (junction 92430)
          (junction 92429) -> (junction 92432)
          (junction 92432) -> Emergency.Doors.Opening1.People_IN.Re_Ready_IN [order 1] : [not(KID_IN|| WOMAN_IN || MAN_IN || FATGUY_IN)]
          (junction 92432) -> (junction 92433) [order 2]
          Emergency.Doors.Opening1.People_IN.Re_Ready_IN -> (junction 92434)
          (junction 92434) -> (junction 92433)
        state Timer_open
          state Set_tmr
            en: Q_op=true;
          state Set
            en:PT_op=2;
            IN_op=true;
          state Counting
            en:ET_op = ET_op + 1;
            Q_op=false;
          (junction 92469) -> Emergency.Doors.Opening1.Timer_open.Set_tmr [order 1] : [ET_op==PT_op]
          Emergency.Doors.Opening1.Timer_open.Set_tmr -> (junction 92470)
          (default) -> Emergency.Doors.Opening1.Timer_open.Set
          Emergency.Doors.Opening1.Timer_open.Counting -> (junction 92469)
          (junction 92469) -> (junction 92470) [order 2]
          Emergency.Doors.Opening1.Timer_open.Set -> (junction 92471)
          (junction 92471) -> Emergency.Doors.Opening1.Timer_open.Counting [order 1] : [ET_op<PT_op]
          (junction 92471) -> (junction 92470) [order 2]
        state Stop_Opening
          en:AP1=false;
          FLAG_OD=true;
          OBS=true;
          IN_op=false;
          ET_op=0;
        state People_OUT
          state Check_People_OUT
            en:
            COUNTER_OUT=false;
          state People_KID_OUT
            en:
            WEIGHT=WEIGHT-30;
            KIDS=KIDS-1;
          state People_WOMAN_OUT
            en:
            WEIGHT=WEIGHT-55;
            WOMEN=WOMEN-1;
          state People_MAN_OUT
            en:
            WEIGHT=WEIGHT-75;
            MEN=MEN-1;
          state People_FATGUY_OUT
            en:
            WEIGHT=WEIGHT-100;
            FATGUYS=FATGUYS-1;
          state Re_Ready_OUT
            en:
            COUNTER_OUT=true;
          (default) -> (junction 92485)
          (junction 92485) -> Emergency.Doors.Opening1.People_OUT.Check_People_OUT [order 1] : [COUNTER_OUT]
          Emergency.Doors.Opening1.People_OUT.Check_People_OUT -> (junction 92486)
          (junction 92486) -> Emergency.Doors.Opening1.People_OUT.People_KID_OUT [order 1] : [KID_OUT && KIDS>0 ]
          Emergency.Doors.Opening1.People_OUT.People_KID_OUT -> (junction 92487)
          (junction 92485) -> (junction 92494) [order 2]
          (junction 92486) -> (junction 92488) [order 2]
          (junction 92487) -> (junction 92489)
          (junction 92488) -> Emergency.Doors.Opening1.People_OUT.People_WOMAN_OUT [order 1] : [WOMAN_OUT && WOMEN>0]
          Emergency.Doors.Opening1.People_OUT.People_WOMAN_OUT -> (junction 92489)
          (junction 92489) -> (junction 92491)
          (junction 92488) -> (junction 92490) [order 2]
          (junction 92490) -> Emergency.Doors.Opening1.People_OUT.People_MAN_OUT [order 1] : [MAN_OUT && MEN>0]
          Emergency.Doors.Opening1.People_OUT.People_MAN_OUT -> (junction 92491)
          (junction 92490) -> (junction 92492) [order 2]
          (junction 92491) -> (junction 92493)
          (junction 92492) -> Emergency.Doors.Opening1.People_OUT.People_FATGUY_OUT [order 1] : [FATGUY_OUT && FATGUYS>0]
          Emergency.Doors.Opening1.People_OUT.People_FATGUY_OUT -> (junction 92493)
          (junction 92492) -> (junction 92495) [order 2]
          (junction 92493) -> (junction 92496)
          (junction 92495) -> (junction 92494)
          (junction 92496) -> (junction 92495)
          (junction 92494) -> (junction 92497)
          (junction 92497) -> Emergency.Doors.Opening1.People_OUT.Re_Ready_OUT [order 1] : [not(KID_OUT || WOMAN_OUT || MAN_OUT || FATGUY_OUT)]
          (junction 92497) -> (junction 92498) [order 2]
          Emergency.Doors.Opening1.People_OUT.Re_Ready_OUT -> (junction 92499)
          (junction 92499) -> (junction 92498)
        state Button_detection
          state Save_energy
            en:
            LL=not(Q_LL);
          state Timer_LL
            state Set_tmr
              en:
              Q_LL=true;
            state Counting
              en:
              ET_LL= ET_LL + 1;
              Q_LL=false;
            state Set
              en:
              IN_LL=true;
              PT_LL=10;
            (junction 92602) -> Emergency.Doors.Opening1.Button_detection.Timer_LL.Set_tmr [order 1] : [ET_LL==PT_LL]
            Emergency.Doors.Opening1.Button_detection.Timer_LL.Set_tmr -> (junction 92603)
            Emergency.Doors.Opening1.Button_detection.Timer_LL.Counting -> (junction 92602)
            (junction 92602) -> (junction 92603) [order 2]
            (default) -> Emergency.Doors.Opening1.Button_detection.Timer_LL.Set
            Emergency.Doors.Opening1.Button_detection.Timer_LL.Set -> (junction 92604)
            (junction 92604) -> Emergency.Doors.Opening1.Button_detection.Timer_LL.Counting [order 1] : [ET_LL<PT_LL]
            (junction 92604) -> (junction 92603) [order 2]
          state BUTTON_DOWN
            state Button_DOWN_1
              en:
              BUTTON_DOWN(2)=true;
              BUT_TEMP=1;
              LPD1=true;
              PUSHED=true;
              UPDATE=false;
              IN_LL=false; ET_LL=0;
            state First_but_1
              en:
              BUT_1=BUT_TEMP;
              FIRST_BUT=false;
            state Button_DOWN_2
              en:
              BUTTON_DOWN(3)=true;
              BUT_TEMP=2;
              LPD2=true;
              PUSHED=true;
              UPDATE=false;
              IN_LL=false; ET_LL=0;
            state First_but_2
              en:
              BUT_1=BUT_TEMP;
              FIRST_BUT=false;
            state Button_DOWN_3
              en:
              BUTTON_DOWN(4)=true;
              BUT_TEMP=3;
              LPD3=true;
              PUSHED=true;
              UPDATE=false;
              IN_LL=false; ET_LL=0;
            state First_but_3
              en:
              BUT_1=BUT_TEMP;
              FIRST_BUT=false;
            (default) -> (junction 92617)
            (junction 92617) -> Emergency.Doors.Opening1.Button_detection.BUTTON_DOWN.Button_DOWN_1 [order 1] : [PD1]
            Emergency.Doors.Opening1.Button_detection.BUTTON_DOWN.Button_DOWN_1 -> (junction 92618)
            (junction 92618) -> Emergency.Doors.Opening1.Button_detection.BUTTON_DOWN.First_but_1 [order 1] : [FIRST_BUT && not(RPC1)]
            Emergency.Doors.Opening1.Button_detection.BUTTON_DOWN.First_but_1 -> (junction 92619)
            (junction 92617) -> (junction 92620) [order 2]
            (junction 92618) -> (junction 92621) [order 2]
            (junction 92619) -> (junction 92622)
            (junction 92621) -> (junction 92620)
            (junction 92622) -> (junction 92621)
            (junction 92620) -> (junction 92623)
            (junction 92623) -> Emergency.Doors.Opening1.Button_detection.BUTTON_DOWN.Button_DOWN_2 [order 1] : [PD2]
            Emergency.Doors.Opening1.Button_detection.BUTTON_DOWN.Button_DOWN_2 -> (junction 92624)
            (junction 92624) -> Emergency.Doors.Opening1.Button_detection.BUTTON_DOWN.First_but_2 [order 1] : [FIRST_BUT && not(RPC2)]
            Emergency.Doors.Opening1.Button_detection.BUTTON_DOWN.First_but_2 -> (junction 92625)
            (junction 92623) -> (junction 92626) [order 2]
            (junction 92624) -> (junction 92627) [order 2]
            (junction 92625) -> (junction 92628)
            (junction 92627) -> (junction 92626)
            (junction 92628) -> (junction 92627)
            (junction 92626) -> (junction 92629)
            (junction 92629) -> Emergency.Doors.Opening1.Button_detection.BUTTON_DOWN.Button_DOWN_3 [order 1] : [PD3]
            Emergency.Doors.Opening1.Button_detection.BUTTON_DOWN.Button_DOWN_3 -> (junction 92630)
            (junction 92630) -> Emergency.Doors.Opening1.Button_detection.BUTTON_DOWN.First_but_3 [order 1] : [FIRST_BUT && not(RPC3)]
            Emergency.Doors.Opening1.Button_detection.BUTTON_DOWN.First_but_3 -> (junction 92631)
            (junction 92629) -> (junction 92632) [order 2]
            (junction 92630) -> (junction 92633) [order 2]
            (junction 92631) -> (junction 92634)
            (junction 92633) -> (junction 92632)
            (junction 92634) -> (junction 92633)
          state BUTTON_CAR
            state Button_CAR_0
              en:
              BUTTON_CAR(1)=true;
              BUT_TEMP=0;
              LPC0=true;
              PUSHED=true;
              UPDATE=false;
              IN_LL=false; ET_LL=0;
            state First_but_0
              en:
              BUT_1=BUT_TEMP;
              FIRST_BUT=false;
            state Button_CAR_1
              en:
              BUTTON_CAR(2)=true;
              BUT_TEMP=1;
              LPC1=true;
              PUSHED=true;
              UPDATE=false;
              IN_LL=false; ET_LL=0;
            state First_but_1
              en:
              BUT_1=BUT_TEMP;
              FIRST_BUT=false;
            state Button_CAR_2
              en:
              BUTTON_CAR(3)=true;
              BUT_TEMP=2;
              LPC2=true;
              PUSHED=true;
              UPDATE=false;
              IN_LL=false; ET_LL=0;
            state First_but_2
              en:
              BUT_1=BUT_TEMP;
              FIRST_BUT=false;
            state Button_CAR_3
              en:
              BUTTON_CAR(4)=true;
              BUT_TEMP=3;
              LPC3=true;
              PUSHED=true;
              UPDATE=false;
              IN_LL=false; ET_LL=0;
            state First_but_3
              en:
              BUT_1=BUT_TEMP;
              FIRST_BUT=false;
            (default) -> (junction 92672)
            (junction 92672) -> Emergency.Doors.Opening1.Button_detection.BUTTON_CAR.Button_CAR_0 [order 1] : [P0]
            Emergency.Doors.Opening1.Button_detection.BUTTON_CAR.Button_CAR_0 -> (junction 92673)
            (junction 92673) -> Emergency.Doors.Opening1.Button_detection.BUTTON_CAR.First_but_0 [order 1] : [FIRST_BUT && not(RPC0)]
            Emergency.Doors.Opening1.Button_detection.BUTTON_CAR.First_but_0 -> (junction 92674)
            (junction 92672) -> (junction 92675) [order 2]
            (junction 92673) -> (junction 92676) [order 2]
            (junction 92674) -> (junction 92677)
            (junction 92676) -> (junction 92675)
            (junction 92677) -> (junction 92676)
            (junction 92675) -> (junction 92680)
            Emergency.Doors.Opening1.Button_detection.BUTTON_CAR.Button_CAR_1 -> (junction 92678)
            (junction 92678) -> Emergency.Doors.Opening1.Button_detection.BUTTON_CAR.First_but_1 [order 1] : [FIRST_BUT && not(RPC1)]
            Emergency.Doors.Opening1.Button_detection.BUTTON_CAR.First_but_1 -> (junction 92679)
            (junction 92678) -> (junction 92682) [order 2]
            (junction 92679) -> (junction 92683)
            (junction 92680) -> Emergency.Doors.Opening1.Button_detection.BUTTON_CAR.Button_CAR_1 [order 1] : [P1]
            (junction 92680) -> (junction 92681) [order 2]
            (junction 92682) -> (junction 92681)
            (junction 92683) -> (junction 92682)
            (junction 92681) -> (junction 92684)
            (junction 92684) -> Emergency.Doors.Opening1.Button_detection.BUTTON_CAR.Button_CAR_2 [order 1] : [P2]
            Emergency.Doors.Opening1.Button_detection.BUTTON_CAR.Button_CAR_2 -> (junction 92685)
            (junction 92685) -> Emergency.Doors.Opening1.Button_detection.BUTTON_CAR.First_but_2 [order 1] : [FIRST_BUT && not(RPC2)]
            Emergency.Doors.Opening1.Button_detection.BUTTON_CAR.First_but_2 -> (junction 92686)
            (junction 92684) -> (junction 92687) [order 2]
            (junction 92685) -> (junction 92688) [order 2]
            (junction 92686) -> (junction 92689)
            (junction 92688) -> (junction 92687)
            (junction 92689) -> (junction 92688)
            (junction 92687) -> (junction 92690)
            (junction 92690) -> Emergency.Doors.Opening1.Button_detection.BUTTON_CAR.Button_CAR_3 [order 1] : [P3]
            Emergency.Doors.Opening1.Button_detection.BUTTON_CAR.Button_CAR_3 -> (junction 92691)
            (junction 92691) -> Emergency.Doors.Opening1.Button_detection.BUTTON_CAR.First_but_3 [order 1] : [FIRST_BUT && not(RPC3)]
            Emergency.Doors.Opening1.Button_detection.BUTTON_CAR.First_but_3 -> (junction 92692)
            (junction 92690) -> (junction 92693) [order 2]
            (junction 92691) -> (junction 92694) [order 2]
            (junction 92692) -> (junction 92695)
            (junction 92694) -> (junction 92693)
            (junction 92695) -> (junction 92694)
          state BUTTON_UP
            state Button_UP_0
              en:
              BUTTON_UP(1)=true;
              BUT_TEMP=0;
              LPS0=true;
              PUSHED=true;
              UPDATE=false;
              IN_LL=false; ET_LL=0;
            state First_but_0
              en:
              BUT_1=BUT_TEMP;
              FIRST_BUT=false;
            state Button_UP_1
              en:
              BUTTON_UP(2)=true;
              BUT_TEMP=1;
              LPS1=true;
              PUSHED=true;
              UPDATE=false;
              IN_LL=false; ET_LL=0;
            state First_but_1
              en:
              BUT_1=BUT_TEMP;
              FIRST_BUT=false;
            state Button_UP_2
              en:
              BUTTON_UP(3)=true;
              BUT_TEMP=2;
              LPS2=true;
              PUSHED=true;
              UPDATE=false;
              IN_LL=false; ET_LL=0;
            state First_but_2
              en:
              BUT_1=BUT_TEMP;
              FIRST_BUT=false;
            (junction 92745) -> Emergency.Doors.Opening1.Button_detection.BUTTON_UP.Button_UP_0 [order 1] : [PS0]
            Emergency.Doors.Opening1.Button_detection.BUTTON_UP.Button_UP_0 -> (junction 92746)
            (junction 92746) -> Emergency.Doors.Opening1.Button_detection.BUTTON_UP.First_but_0 [order 1] : [FIRST_BUT && not(RPC0)]
            Emergency.Doors.Opening1.Button_detection.BUTTON_UP.First_but_0 -> (junction 92747)
            (default) -> (junction 92745)
            (junction 92745) -> (junction 92750) [order 2]
            (junction 92746) -> (junction 92748) [order 2]
            (junction 92747) -> (junction 92749)
            (junction 92749) -> (junction 92748)
            (junction 92748) -> (junction 92750)
            (junction 92750) -> (junction 92751)
            (junction 92751) -> Emergency.Doors.Opening1.Button_detection.BUTTON_UP.Button_UP_1 [order 1] : [PS1]
            Emergency.Doors.Opening1.Button_detection.BUTTON_UP.Button_UP_1 -> (junction 92752)
            (junction 92752) -> Emergency.Doors.Opening1.Button_detection.BUTTON_UP.First_but_1 [order 1] : [FIRST_BUT && not(RPC1)]
            Emergency.Doors.Opening1.Button_detection.BUTTON_UP.First_but_1 -> (junction 92753)
            (junction 92751) -> (junction 92754) [order 2]
            (junction 92752) -> (junction 92755) [order 2]
            (junction 92753) -> (junction 92756)
            (junction 92755) -> (junction 92754)
            (junction 92756) -> (junction 92755)
            (junction 92754) -> (junction 92758)
            Emergency.Doors.Opening1.Button_detection.BUTTON_UP.First_but_2 -> (junction 92757)
            (junction 92757) -> (junction 92762)
            (junction 92758) -> Emergency.Doors.Opening1.Button_detection.BUTTON_UP.Button_UP_2 [order 1] : [PS2]
            Emergency.Doors.Opening1.Button_detection.BUTTON_UP.Button_UP_2 -> (junction 92759)
            (junction 92759) -> Emergency.Doors.Opening1.Button_detection.BUTTON_UP.First_but_2 [order 1] : [FIRST_BUT && not(RPC2)]
            (junction 92758) -> (junction 92760) [order 2]
            (junction 92759) -> (junction 92761) [order 2]
            (junction 92761) -> (junction 92760)
            (junction 92762) -> (junction 92761)
          state Max_Min_assignment
            state Min_but
              en:
              BUTTON=MIN_BUT;
            state Max_but
              en:
              BUTTON=MAX_BUT;
            state First_but
              en:
              BUTTON=BUT_1;
            state Max_but1
              en:
              MAX_BUT=2;
            state Max_but2
              en:
              MAX_BUT=1;
            state Max_but3
              en:
              MAX_BUT=0;
            state Min_but1
              en:
              MIN_BUT=1;
            state Min_but2
              en:
              MIN_BUT=2;
            state Min_but3
              en:
              MIN_BUT=3;
            state MAX
              en:
              MAX_BUT=BUT_TEMP;
            state MIN
              en:
              MIN_BUT=BUT_TEMP;
            state Updating_button_0
              en:
              BUTTON=MAX_BUT;
            state Updating_button_1
              en:
              BUTTON=MIN_BUT;
            (junction 92800) -> Emergency.Doors.Opening1.Button_detection.Max_Min_assignment.Min_but [order 1] : [(MAX_BUT-FLOOR)>(FLOOR-MIN_BUT)]
            Emergency.Doors.Opening1.Button_detection.Max_Min_assignment.Min_but -> (junction 92801)
            (junction 92802) -> (junction 92800) [order 1] : [not(FLAG_STOP) && MOTION==2 && FLAG==3]
            (default) -> (junction 92802)
            (junction 92800) -> (junction 92803) [order 2]
            (junction 92801) -> (junction 92804)
            (junction 92802) -> (junction 92805) [order 2]
            (junction 92803) -> Emergency.Doors.Opening1.Button_detection.Max_Min_assignment.Max_but [order 1] : [(MAX_BUT-FLOOR)<(FLOOR-MIN_BUT)]
            Emergency.Doors.Opening1.Button_detection.Max_Min_assignment.Max_but -> (junction 92804)
            (junction 92803) -> Emergency.Doors.Opening1.Button_detection.Max_Min_assignment.First_but [order 2]
            (junction 92804) -> (junction 92807)
            Emergency.Doors.Opening1.Button_detection.Max_Min_assignment.First_but -> (junction 92806)
            (junction 92806) -> (junction 92805)
            (junction 92807) -> (junction 92806)
            (junction 92805) -> (junction 92808)
            (junction 92809) -> (junction 92810) [order 1] : [MOTION==0]
                | {MOTION=1;
                | UPDATE=true;}
            (junction 92810) -> Emergency.Doors.Opening1.Button_detection.Max_Min_assignment.Max_but1 [order 1] : [BUTTON_UP(2)]
            Emergency.Doors.Opening1.Button_detection.Max_Min_assignment.Max_but1 -> (junction 92811)
            (junction 92808) -> (junction 92809) [order 1] : [BUTTON==FLOOR && EXTEND]
                | {EXTEND=false;}
            (junction 92808) -> (junction 92822) [order 2]
            (junction 92809) -> (junction 92814) [order 2]
            (junction 92810) -> (junction 92812) [order 2]
            (junction 92811) -> (junction 92813)
            (junction 92812) -> Emergency.Doors.Opening1.Button_detection.Max_Min_assignment.Max_but2 [order 1] : [BUTTON_UP(1)]
            Emergency.Doors.Opening1.Button_detection.Max_Min_assignment.Max_but2 -> (junction 92813)
            (junction 92812) -> Emergency.Doors.Opening1.Button_detection.Max_Min_assignment.Max_but3 [order 2]
            (junction 92813) -> (junction 92816)
            Emergency.Doors.Opening1.Button_detection.Max_Min_assignment.Max_but3 -> (junction 92815)
            (junction 92815) -> (junction 92814)
            (junction 92816) -> (junction 92815)
            (junction 92814) -> (junction 92817)
            (junction 92817) -> (junction 92818) [order 1] : [MOTION==1]
                | {MOTION=0;
                | UPDATE=true;}
            (junction 92818) -> Emergency.Doors.Opening1.Button_detection.Max_Min_assignment.Min_but1 [order 1] : [BUTTON_DOWN(1)]
            Emergency.Doors.Opening1.Button_detection.Max_Min_assignment.Min_but1 -> (junction 92819)
            (junction 92817) -> (junction 92823) [order 2]
            (junction 92818) -> (junction 92820) [order 2]
            (junction 92819) -> (junction 92821)
            (junction 92820) -> Emergency.Doors.Opening1.Button_detection.Max_Min_assignment.Min_but2 [order 1] : [BUTTON_DOWN(2)]
            Emergency.Doors.Opening1.Button_detection.Max_Min_assignment.Min_but2 -> (junction 92821)
            (junction 92820) -> Emergency.Doors.Opening1.Button_detection.Max_Min_assignment.Min_but3 [order 2]
            (junction 92821) -> (junction 92825)
            Emergency.Doors.Opening1.Button_detection.Max_Min_assignment.Min_but3 -> (junction 92824)
            (junction 92823) -> (junction 92822)
            (junction 92824) -> (junction 92823)
            (junction 92825) -> (junction 92824)
            (junction 92822) -> (junction 92827)
            Emergency.Doors.Opening1.Button_detection.Max_Min_assignment.MAX -> (junction 92826)
            (junction 92827) -> (junction 92828) [order 1] : [PUSHED]
            (junction 92828) -> (junction 92829) [order 1] : [not(BUT_TEMP==FLOOR) || not(MOTION==2)]
            (junction 92829) -> Emergency.Doors.Opening1.Button_detection.Max_Min_assignment.MAX [order 1] : [MAX_BUT<BUT_TEMP && not(UPDATE)]
            (junction 92826) -> (junction 92831)
            (junction 92827) -> (junction 92841) [order 2]
            (junction 92828) -> (junction 92834) [order 2]
            (junction 92829) -> (junction 92830) [order 2]
            (junction 92831) -> (junction 92830)
            (junction 92830) -> (junction 92832)
            (junction 92832) -> Emergency.Doors.Opening1.Button_detection.Max_Min_assignment.MIN [order 1] : [MIN_BUT>BUT_TEMP && not(UPDATE)]
            Emergency.Doors.Opening1.Button_detection.Max_Min_assignment.MIN -> (junction 92833)
            (junction 92832) -> (junction 92835) [order 2]
            (junction 92833) -> (junction 92836)
            (junction 92835) -> (junction 92834)
            (junction 92836) -> (junction 92835)
            (junction 92834) -> (junction 92837)
            (junction 92837) -> Emergency.Doors.Opening1.Button_detection.Max_Min_assignment.Updating_button_0 [order 1] : [MOTION==0]
            Emergency.Doors.Opening1.Button_detection.Max_Min_assignment.Updating_button_0 -> (junction 92838)
            (junction 92837) -> (junction 92839) [order 2]
            (junction 92838) -> (junction 92840)
            (junction 92839) -> Emergency.Doors.Opening1.Button_detection.Max_Min_assignment.Updating_button_1 [order 1] : [MOTION==1]
            Emergency.Doors.Opening1.Button_detection.Max_Min_assignment.Updating_button_1 -> (junction 92840)
            (junction 92839) -> (junction 92842) [order 2]
            (junction 92840) -> (junction 92843)
            (junction 92842) -> (junction 92841)
            (junction 92843) -> (junction 92842)
          state GoTo_PositionControl
            en:
            BUTTON=BUT_TEMP;
            FLAG=2;
          state Emergency
            en:
            FLAG_EMG=true;
            FLAG=4;
          state Timer_EME
            state Set_tmr
              en:
              Q_EME=true;
            state Counting
              en:
              ET_EME= ET_EME + 1;
              Q_EME=false;
            state Set
              en:
              IN_EME=true;
              PT_EME=3;
            (junction 92933) -> Emergency.Doors.Opening1.Button_detection.Timer_EME.Set_tmr [order 1] : [ET_EME==PT_EME]
            Emergency.Doors.Opening1.Button_detection.Timer_EME.Set_tmr -> (junction 92934)
            Emergency.Doors.Opening1.Button_detection.Timer_EME.Counting -> (junction 92933)
            (junction 92933) -> (junction 92934) [order 2]
            (default) -> Emergency.Doors.Opening1.Button_detection.Timer_EME.Set
            Emergency.Doors.Opening1.Button_detection.Timer_EME.Set -> (junction 92935)
            (junction 92935) -> Emergency.Doors.Opening1.Button_detection.Timer_EME.Counting [order 1] : [ET_EME<PT_EME]
            (junction 92935) -> (junction 92934) [order 2]
          state Not_Emergency
            en:
            IN_EME=false;
            ET_EME=0;
          state SwitchingOFF_LEDs
            en:
            LPD3=false;
            LPD2=false;
            LPS2=false;
            LPD1=false;
            LPS1=false;
            LPS0=false;
          (default) -> (junction 92534)
          (junction 92534) -> (junction 92535) [order 1] : [FLAG==1 && not(PUSHED)]
              | {BUTTON=FLOOR;
              | BUT_TEMP=BUTTON;
              | BUT_1=FLOOR;}
          (junction 92535) -> Emergency.Doors.Opening1.Button_detection.Timer_LL [order 1] : [not(FLAG_STOP)]
          Emergency.Doors.Opening1.Button_detection.Timer_LL -> Emergency.Doors.Opening1.Button_detection.Save_energy
          Emergency.Doors.Opening1.Button_detection.Save_energy -> (junction 92536)
          (junction 92534) -> (junction 92537) [order 2]
          (junction 92535) -> (junction 92538) [order 2]
          (junction 92536) -> (junction 92539)
          (junction 92538) -> (junction 92537)
          (junction 92539) -> (junction 92538)
          (junction 92537) -> Emergency.Doors.Opening1.Button_detection.BUTTON_CAR
          Emergency.Doors.Opening1.Button_detection.BUTTON_UP -> Emergency.Doors.Opening1.Button_detection.BUTTON_DOWN
          Emergency.Doors.Opening1.Button_detection.BUTTON_DOWN -> Emergency.Doors.Opening1.Button_detection.Max_Min_assignment
          Emergency.Doors.Opening1.Button_detection.Max_Min_assignment -> (junction 92540)
          Emergency.Doors.Opening1.Button_detection.BUTTON_CAR -> Emergency.Doors.Opening1.Button_detection.BUTTON_UP
          (junction 92540) -> (junction 92542)
          (junction 92542) -> (junction 92541)
          (junction 92541) -> (junction 92543)
          (junction 92543) -> (junction 92544) [order 1] : [FLAG==1]
          (junction 92544) -> Emergency.Doors.Opening1.Button_detection.GoTo_PositionControl [order 1] : [PUSHED]
          Emergency.Doors.Opening1.Button_detection.GoTo_PositionControl -> (junction 92545)
          (junction 92543) -> (junction 92555) [order 2]
          (junction 92544) -> (junction 92546) [order 2]
          (junction 92545) -> (junction 92547)
          (junction 92547) -> (junction 92546)
          (junction 92546) -> (junction 92549)
          Emergency.Doors.Opening1.Button_detection.Emergency -> (junction 92548)
          (junction 92549) -> Emergency.Doors.Opening1.Button_detection.Timer_EME [order 1] : [STOP]
              | {IN_LL=false; ET_LL=0;FLAG=1;}
          Emergency.Doors.Opening1.Button_detection.Timer_EME -> (junction 92550)
          (junction 92550) -> Emergency.Doors.Opening1.Button_detection.Emergency [order 1] : [Q_EME]
          (junction 92548) -> (junction 92552)
          (junction 92549) -> Emergency.Doors.Opening1.Button_detection.Not_Emergency [order 2]
          (junction 92550) -> (junction 92551) [order 2]
          (junction 92552) -> (junction 92551)
          (junction 92551) -> (junction 92554)
          Emergency.Doors.Opening1.Button_detection.Not_Emergency -> (junction 92554)
          Emergency.Doors.Opening1.Button_detection.SwitchingOFF_LEDs -> (junction 92553)
          (junction 92554) -> Emergency.Doors.Opening1.Button_detection.SwitchingOFF_LEDs [order 1] : [FLAG_STOP && FLAG==2]
          (junction 92553) -> (junction 92557)
          (junction 92554) -> (junction 92556) [order 2]
          (junction 92556) -> (junction 92555)
          (junction 92557) -> (junction 92556)
        state Button_detection1
          state Save_energy
            en:
            LL=not(Q_LL);
          state Timer_LL
            state Set_tmr
              en:
              Q_LL=true;
            state Counting
              en:
              ET_LL= ET_LL + 1;
              Q_LL=false;
            state Set
              en:
              IN_LL=true;
              PT_LL=10;
            (junction 93018) -> Emergency.Doors.Opening1.Button_detection1.Timer_LL.Set_tmr [order 1] : [ET_LL==PT_LL]
            Emergency.Doors.Opening1.Button_detection1.Timer_LL.Set_tmr -> (junction 93019)
            Emergency.Doors.Opening1.Button_detection1.Timer_LL.Counting -> (junction 93018)
            (junction 93018) -> (junction 93019) [order 2]
            (default) -> Emergency.Doors.Opening1.Button_detection1.Timer_LL.Set
            Emergency.Doors.Opening1.Button_detection1.Timer_LL.Set -> (junction 93020)
            (junction 93020) -> Emergency.Doors.Opening1.Button_detection1.Timer_LL.Counting [order 1] : [ET_LL<PT_LL]
            (junction 93020) -> (junction 93019) [order 2]
          state BUTTON_DOWN
            state Button_DOWN_1
              en:
              BUTTON_DOWN(2)=true;
              BUT_TEMP=1;
              LPD1=true;
              PUSHED=true;
              UPDATE=false;
              IN_LL=false; ET_LL=0;
            state First_but_1
              en:
              BUT_1=BUT_TEMP;
              FIRST_BUT=false;
            state Button_DOWN_2
              en:
              BUTTON_DOWN(3)=true;
              BUT_TEMP=2;
              LPD2=true;
              PUSHED=true;
              UPDATE=false;
              IN_LL=false; ET_LL=0;
            state First_but_2
              en:
              BUT_1=BUT_TEMP;
              FIRST_BUT=false;
            state Button_DOWN_3
              en:
              BUTTON_DOWN(4)=true;
              BUT_TEMP=3;
              LPD3=true;
              PUSHED=true;
              UPDATE=false;
              IN_LL=false; ET_LL=0;
            state First_but_3
              en:
              BUT_1=BUT_TEMP;
              FIRST_BUT=false;
            (default) -> (junction 93033)
            (junction 93033) -> Emergency.Doors.Opening1.Button_detection1.BUTTON_DOWN.Button_DOWN_1 [order 1] : [PD1]
            Emergency.Doors.Opening1.Button_detection1.BUTTON_DOWN.Button_DOWN_1 -> (junction 93034)
            (junction 93034) -> Emergency.Doors.Opening1.Button_detection1.BUTTON_DOWN.First_but_1 [order 1] : [FIRST_BUT && not(RPC1)]
            Emergency.Doors.Opening1.Button_detection1.BUTTON_DOWN.First_but_1 -> (junction 93035)
            (junction 93033) -> (junction 93036) [order 2]
            (junction 93034) -> (junction 93037) [order 2]
            (junction 93035) -> (junction 93038)
            (junction 93037) -> (junction 93036)
            (junction 93038) -> (junction 93037)
            (junction 93036) -> (junction 93039)
            (junction 93039) -> Emergency.Doors.Opening1.Button_detection1.BUTTON_DOWN.Button_DOWN_2 [order 1] : [PD2]
            Emergency.Doors.Opening1.Button_detection1.BUTTON_DOWN.Button_DOWN_2 -> (junction 93040)
            (junction 93040) -> Emergency.Doors.Opening1.Button_detection1.BUTTON_DOWN.First_but_2 [order 1] : [FIRST_BUT && not(RPC2)]
            Emergency.Doors.Opening1.Button_detection1.BUTTON_DOWN.First_but_2 -> (junction 93041)
            (junction 93039) -> (junction 93042) [order 2]
            (junction 93040) -> (junction 93043) [order 2]
            (junction 93041) -> (junction 93044)
            (junction 93043) -> (junction 93042)
            (junction 93044) -> (junction 93043)
            (junction 93042) -> (junction 93045)
            (junction 93045) -> Emergency.Doors.Opening1.Button_detection1.BUTTON_DOWN.Button_DOWN_3 [order 1] : [PD3]
            Emergency.Doors.Opening1.Button_detection1.BUTTON_DOWN.Button_DOWN_3 -> (junction 93046)
            (junction 93046) -> Emergency.Doors.Opening1.Button_detection1.BUTTON_DOWN.First_but_3 [order 1] : [FIRST_BUT && not(RPC3)]
            Emergency.Doors.Opening1.Button_detection1.BUTTON_DOWN.First_but_3 -> (junction 93047)
            (junction 93045) -> (junction 93048) [order 2]
            (junction 93046) -> (junction 93049) [order 2]
            (junction 93047) -> (junction 93050)
            (junction 93049) -> (junction 93048)
            (junction 93050) -> (junction 93049)
          state BUTTON_CAR
            state Button_CAR_0
              en:
              BUTTON_CAR(1)=true;
              BUT_TEMP=0;
              LPC0=true;
              PUSHED=true;
              UPDATE=false;
              IN_LL=false; ET_LL=0;
            state First_but_0
              en:
              BUT_1=BUT_TEMP;
              FIRST_BUT=false;
            state Button_CAR_1
              en:
              BUTTON_CAR(2)=true;
              BUT_TEMP=1;
              LPC1=true;
              PUSHED=true;
              UPDATE=false;
              IN_LL=false; ET_LL=0;
            state First_but_1
              en:
              BUT_1=BUT_TEMP;
              FIRST_BUT=false;
            state Button_CAR_2
              en:
              BUTTON_CAR(3)=true;
              BUT_TEMP=2;
              LPC2=true;
              PUSHED=true;
              UPDATE=false;
              IN_LL=false; ET_LL=0;
            state First_but_2
              en:
              BUT_1=BUT_TEMP;
              FIRST_BUT=false;
            state Button_CAR_3
              en:
              BUTTON_CAR(4)=true;
              BUT_TEMP=3;
              LPC3=true;
              PUSHED=true;
              UPDATE=false;
              IN_LL=false; ET_LL=0;
            state First_but_3
              en:
              BUT_1=BUT_TEMP;
              FIRST_BUT=false;
            (default) -> (junction 93088)
            (junction 93088) -> Emergency.Doors.Opening1.Button_detection1.BUTTON_CAR.Button_CAR_0 [order 1] : [P0]
            Emergency.Doors.Opening1.Button_detection1.BUTTON_CAR.Button_CAR_0 -> (junction 93089)
            (junction 93089) -> Emergency.Doors.Opening1.Button_detection1.BUTTON_CAR.First_but_0 [order 1] : [FIRST_BUT && not(RPC0)]
            Emergency.Doors.Opening1.Button_detection1.BUTTON_CAR.First_but_0 -> (junction 93090)
            (junction 93088) -> (junction 93091) [order 2]
            (junction 93089) -> (junction 93092) [order 2]
            (junction 93090) -> (junction 93093)
            (junction 93092) -> (junction 93091)
            (junction 93093) -> (junction 93092)
            (junction 93091) -> (junction 93096)
            Emergency.Doors.Opening1.Button_detection1.BUTTON_CAR.Button_CAR_1 -> (junction 93094)
            (junction 93094) -> Emergency.Doors.Opening1.Button_detection1.BUTTON_CAR.First_but_1 [order 1] : [FIRST_BUT && not(RPC1)]
            Emergency.Doors.Opening1.Button_detection1.BUTTON_CAR.First_but_1 -> (junction 93095)
            (junction 93094) -> (junction 93098) [order 2]
            (junction 93095) -> (junction 93099)
            (junction 93096) -> Emergency.Doors.Opening1.Button_detection1.BUTTON_CAR.Button_CAR_1 [order 1] : [P1]
            (junction 93096) -> (junction 93097) [order 2]
            (junction 93098) -> (junction 93097)
            (junction 93099) -> (junction 93098)
            (junction 93097) -> (junction 93100)
            (junction 93100) -> Emergency.Doors.Opening1.Button_detection1.BUTTON_CAR.Button_CAR_2 [order 1] : [P2]
            Emergency.Doors.Opening1.Button_detection1.BUTTON_CAR.Button_CAR_2 -> (junction 93101)
            (junction 93101) -> Emergency.Doors.Opening1.Button_detection1.BUTTON_CAR.First_but_2 [order 1] : [FIRST_BUT && not(RPC2)]
            Emergency.Doors.Opening1.Button_detection1.BUTTON_CAR.First_but_2 -> (junction 93102)
            (junction 93100) -> (junction 93103) [order 2]
            (junction 93101) -> (junction 93104) [order 2]
            (junction 93102) -> (junction 93105)
            (junction 93104) -> (junction 93103)
            (junction 93105) -> (junction 93104)
            (junction 93103) -> (junction 93106)
            (junction 93106) -> Emergency.Doors.Opening1.Button_detection1.BUTTON_CAR.Button_CAR_3 [order 1] : [P3]
            Emergency.Doors.Opening1.Button_detection1.BUTTON_CAR.Button_CAR_3 -> (junction 93107)
            (junction 93107) -> Emergency.Doors.Opening1.Button_detection1.BUTTON_CAR.First_but_3 [order 1] : [FIRST_BUT && not(RPC3)]
            Emergency.Doors.Opening1.Button_detection1.BUTTON_CAR.First_but_3 -> (junction 93108)
            (junction 93106) -> (junction 93109) [order 2]
            (junction 93107) -> (junction 93110) [order 2]
            (junction 93108) -> (junction 93111)
            (junction 93110) -> (junction 93109)
            (junction 93111) -> (junction 93110)
          state BUTTON_UP
            state Button_UP_0
              en:
              BUTTON_UP(1)=true;
              BUT_TEMP=0;
              LPS0=true;
              PUSHED=true;
              UPDATE=false;
              IN_LL=false; ET_LL=0;
            state First_but_0
              en:
              BUT_1=BUT_TEMP;
              FIRST_BUT=false;
            state Button_UP_1
              en:
              BUTTON_UP(2)=true;
              BUT_TEMP=1;
              LPS1=true;
              PUSHED=true;
              UPDATE=false;
              IN_LL=false; ET_LL=0;
            state First_but_1
              en:
              BUT_1=BUT_TEMP;
              FIRST_BUT=false;
            state Button_UP_2
              en:
              BUTTON_UP(3)=true;
              BUT_TEMP=2;
              LPS2=true;
              PUSHED=true;
              UPDATE=false;
              IN_LL=false; ET_LL=0;
            state First_but_2
              en:
              BUT_1=BUT_TEMP;
              FIRST_BUT=false;
            (junction 93161) -> Emergency.Doors.Opening1.Button_detection1.BUTTON_UP.Button_UP_0 [order 1] : [PS0]
            Emergency.Doors.Opening1.Button_detection1.BUTTON_UP.Button_UP_0 -> (junction 93162)
            (junction 93162) -> Emergency.Doors.Opening1.Button_detection1.BUTTON_UP.First_but_0 [order 1] : [FIRST_BUT && not(RPC0)]
            Emergency.Doors.Opening1.Button_detection1.BUTTON_UP.First_but_0 -> (junction 93163)
            (default) -> (junction 93161)
            (junction 93161) -> (junction 93166) [order 2]
            (junction 93162) -> (junction 93164) [order 2]
            (junction 93163) -> (junction 93165)
            (junction 93165) -> (junction 93164)
            (junction 93164) -> (junction 93166)
            (junction 93166) -> (junction 93167)
            (junction 93167) -> Emergency.Doors.Opening1.Button_detection1.BUTTON_UP.Button_UP_1 [order 1] : [PS1]
            Emergency.Doors.Opening1.Button_detection1.BUTTON_UP.Button_UP_1 -> (junction 93168)
            (junction 93168) -> Emergency.Doors.Opening1.Button_detection1.BUTTON_UP.First_but_1 [order 1] : [FIRST_BUT && not(RPC1)]
            Emergency.Doors.Opening1.Button_detection1.BUTTON_UP.First_but_1 -> (junction 93169)
            (junction 93167) -> (junction 93170) [order 2]
            (junction 93168) -> (junction 93171) [order 2]
            (junction 93169) -> (junction 93172)
            (junction 93171) -> (junction 93170)
            (junction 93172) -> (junction 93171)
            (junction 93170) -> (junction 93174)
            Emergency.Doors.Opening1.Button_detection1.BUTTON_UP.First_but_2 -> (junction 93173)
            (junction 93173) -> (junction 93178)
            (junction 93174) -> Emergency.Doors.Opening1.Button_detection1.BUTTON_UP.Button_UP_2 [order 1] : [PS2]
            Emergency.Doors.Opening1.Button_detection1.BUTTON_UP.Button_UP_2 -> (junction 93175)
            (junction 93175) -> Emergency.Doors.Opening1.Button_detection1.BUTTON_UP.First_but_2 [order 1] : [FIRST_BUT && not(RPC2)]
            (junction 93174) -> (junction 93176) [order 2]
            (junction 93175) -> (junction 93177) [order 2]
            (junction 93177) -> (junction 93176)
            (junction 93178) -> (junction 93177)
          state Max_Min_assignment
            state Min_but
              en:
              BUTTON=MIN_BUT;
            state Max_but
              en:
              BUTTON=MAX_BUT;
            state First_but
              en:
              BUTTON=BUT_1;
            state Max_but1
              en:
              MAX_BUT=2;
            state Max_but2
              en:
              MAX_BUT=1;
            state Max_but3
              en:
              MAX_BUT=0;
            state Min_but1
              en:
              MIN_BUT=1;
            state Min_but2
              en:
              MIN_BUT=2;
            state Min_but3
              en:
              MIN_BUT=3;
            state MAX
              en:
              MAX_BUT=BUT_TEMP;
            state MIN
              en:
              MIN_BUT=BUT_TEMP;
            state Updating_button_0
              en:
              BUTTON=MAX_BUT;
            state Updating_button_1
              en:
              BUTTON=MIN_BUT;
            (junction 93216) -> Emergency.Doors.Opening1.Button_detection1.Max_Min_assignment.Min_but [order 1] : [(MAX_BUT-FLOOR)>(FLOOR-MIN_BUT)]
            Emergency.Doors.Opening1.Button_detection1.Max_Min_assignment.Min_but -> (junction 93217)
            (junction 93218) -> (junction 93216) [order 1] : [not(FLAG_STOP) && MOTION==2 && FLAG==3]
            (default) -> (junction 93218)
            (junction 93216) -> (junction 93219) [order 2]
            (junction 93217) -> (junction 93220)
            (junction 93218) -> (junction 93221) [order 2]
            (junction 93219) -> Emergency.Doors.Opening1.Button_detection1.Max_Min_assignment.Max_but [order 1] : [(MAX_BUT-FLOOR)<(FLOOR-MIN_BUT)]
            Emergency.Doors.Opening1.Button_detection1.Max_Min_assignment.Max_but -> (junction 93220)
            (junction 93219) -> Emergency.Doors.Opening1.Button_detection1.Max_Min_assignment.First_but [order 2]
            (junction 93220) -> (junction 93223)
            Emergency.Doors.Opening1.Button_detection1.Max_Min_assignment.First_but -> (junction 93222)
            (junction 93222) -> (junction 93221)
            (junction 93223) -> (junction 93222)
            (junction 93221) -> (junction 93224)
            (junction 93225) -> (junction 93226) [order 1] : [MOTION==0]
                | {MOTION=1;
                | UPDATE=true;}
            (junction 93226) -> Emergency.Doors.Opening1.Button_detection1.Max_Min_assignment.Max_but1 [order 1] : [BUTTON_UP(2)]
            Emergency.Doors.Opening1.Button_detection1.Max_Min_assignment.Max_but1 -> (junction 93227)
            (junction 93224) -> (junction 93225) [order 1] : [BUTTON==FLOOR && EXTEND]
                | {EXTEND=false;}
            (junction 93224) -> (junction 93238) [order 2]
            (junction 93225) -> (junction 93230) [order 2]
            (junction 93226) -> (junction 93228) [order 2]
            (junction 93227) -> (junction 93229)
            (junction 93228) -> Emergency.Doors.Opening1.Button_detection1.Max_Min_assignment.Max_but2 [order 1] : [BUTTON_UP(1)]
            Emergency.Doors.Opening1.Button_detection1.Max_Min_assignment.Max_but2 -> (junction 93229)
            (junction 93228) -> Emergency.Doors.Opening1.Button_detection1.Max_Min_assignment.Max_but3 [order 2]
            (junction 93229) -> (junction 93232)
            Emergency.Doors.Opening1.Button_detection1.Max_Min_assignment.Max_but3 -> (junction 93231)
            (junction 93231) -> (junction 93230)
            (junction 93232) -> (junction 93231)
            (junction 93230) -> (junction 93233)
            (junction 93233) -> (junction 93234) [order 1] : [MOTION==1]
                | {MOTION=0;
                | UPDATE=true;}
            (junction 93234) -> Emergency.Doors.Opening1.Button_detection1.Max_Min_assignment.Min_but1 [order 1] : [BUTTON_DOWN(1)]
            Emergency.Doors.Opening1.Button_detection1.Max_Min_assignment.Min_but1 -> (junction 93235)
            (junction 93233) -> (junction 93239) [order 2]
            (junction 93234) -> (junction 93236) [order 2]
            (junction 93235) -> (junction 93237)
            (junction 93236) -> Emergency.Doors.Opening1.Button_detection1.Max_Min_assignment.Min_but2 [order 1] : [BUTTON_DOWN(2)]
            Emergency.Doors.Opening1.Button_detection1.Max_Min_assignment.Min_but2 -> (junction 93237)
            (junction 93236) -> Emergency.Doors.Opening1.Button_detection1.Max_Min_assignment.Min_but3 [order 2]
            (junction 93237) -> (junction 93241)
            Emergency.Doors.Opening1.Button_detection1.Max_Min_assignment.Min_but3 -> (junction 93240)
            (junction 93239) -> (junction 93238)
            (junction 93240) -> (junction 93239)
            (junction 93241) -> (junction 93240)
            (junction 93238) -> (junction 93243)
            Emergency.Doors.Opening1.Button_detection1.Max_Min_assignment.MAX -> (junction 93242)
            (junction 93243) -> (junction 93244) [order 1] : [PUSHED]
            (junction 93244) -> (junction 93245) [order 1] : [not(BUT_TEMP==FLOOR) || not(MOTION==2)]
            (junction 93245) -> Emergency.Doors.Opening1.Button_detection1.Max_Min_assignment.MAX [order 1] : [MAX_BUT<BUT_TEMP && not(UPDATE)]
            (junction 93242) -> (junction 93247)
            (junction 93243) -> (junction 93257) [order 2]
            (junction 93244) -> (junction 93250) [order 2]
            (junction 93245) -> (junction 93246) [order 2]
            (junction 93247) -> (junction 93246)
            (junction 93246) -> (junction 93248)
            (junction 93248) -> Emergency.Doors.Opening1.Button_detection1.Max_Min_assignment.MIN [order 1] : [MIN_BUT>BUT_TEMP && not(UPDATE)]
            Emergency.Doors.Opening1.Button_detection1.Max_Min_assignment.MIN -> (junction 93249)
            (junction 93248) -> (junction 93251) [order 2]
            (junction 93249) -> (junction 93252)
            (junction 93251) -> (junction 93250)
            (junction 93252) -> (junction 93251)
            (junction 93250) -> (junction 93253)
            (junction 93253) -> Emergency.Doors.Opening1.Button_detection1.Max_Min_assignment.Updating_button_0 [order 1] : [MOTION==0]
            Emergency.Doors.Opening1.Button_detection1.Max_Min_assignment.Updating_button_0 -> (junction 93254)
            (junction 93253) -> (junction 93255) [order 2]
            (junction 93254) -> (junction 93256)
            (junction 93255) -> Emergency.Doors.Opening1.Button_detection1.Max_Min_assignment.Updating_button_1 [order 1] : [MOTION==1]
            Emergency.Doors.Opening1.Button_detection1.Max_Min_assignment.Updating_button_1 -> (junction 93256)
            (junction 93255) -> (junction 93258) [order 2]
            (junction 93256) -> (junction 93259)
            (junction 93258) -> (junction 93257)
            (junction 93259) -> (junction 93258)
          state GoTo_PositionControl
            en:
            BUTTON=BUT_TEMP;
            FLAG=2;
          state Emergency
            en:
            FLAG_EMG=true;
            FLAG=4;
          state Timer_EME
            state Set_tmr
              en:
              Q_EME=true;
            state Counting
              en:
              ET_EME= ET_EME + 1;
              Q_EME=false;
            state Set
              en:
              IN_EME=true;
              PT_EME=3;
            (junction 93349) -> Emergency.Doors.Opening1.Button_detection1.Timer_EME.Set_tmr [order 1] : [ET_EME==PT_EME]
            Emergency.Doors.Opening1.Button_detection1.Timer_EME.Set_tmr -> (junction 93350)
            Emergency.Doors.Opening1.Button_detection1.Timer_EME.Counting -> (junction 93349)
            (junction 93349) -> (junction 93350) [order 2]
            (default) -> Emergency.Doors.Opening1.Button_detection1.Timer_EME.Set
            Emergency.Doors.Opening1.Button_detection1.Timer_EME.Set -> (junction 93351)
            (junction 93351) -> Emergency.Doors.Opening1.Button_detection1.Timer_EME.Counting [order 1] : [ET_EME<PT_EME]
            (junction 93351) -> (junction 93350) [order 2]
          state Not_Emergency
            en:
            IN_EME=false;
            ET_EME=0;
          state SwitchingOFF_LEDs
            en:
            LPD3=false;
            LPD2=false;
            LPS2=false;
            LPD1=false;
            LPS1=false;
            LPS0=false;
          (default) -> (junction 92950)
          (junction 92950) -> (junction 92951) [order 1] : [FLAG==1 && not(PUSHED)]
              | {BUTTON=FLOOR;
              | BUT_TEMP=BUTTON;
              | BUT_1=FLOOR;}
          (junction 92951) -> Emergency.Doors.Opening1.Button_detection1.Timer_LL [order 1] : [not(FLAG_STOP)]
          Emergency.Doors.Opening1.Button_detection1.Save_energy -> (junction 92952)
          Emergency.Doors.Opening1.Button_detection1.Timer_LL -> Emergency.Doors.Opening1.Button_detection1.Save_energy
          (junction 92951) -> (junction 92954) [order 2]
          (junction 92950) -> (junction 92953) [order 2]
          (junction 92952) -> (junction 92955)
          (junction 92954) -> (junction 92953)
          (junction 92955) -> (junction 92954)
          (junction 92953) -> Emergency.Doors.Opening1.Button_detection1.BUTTON_CAR
          Emergency.Doors.Opening1.Button_detection1.BUTTON_UP -> Emergency.Doors.Opening1.Button_detection1.BUTTON_DOWN
          Emergency.Doors.Opening1.Button_detection1.BUTTON_DOWN -> Emergency.Doors.Opening1.Button_detection1.Max_Min_assignment
          Emergency.Doors.Opening1.Button_detection1.Max_Min_assignment -> (junction 92956)
          Emergency.Doors.Opening1.Button_detection1.BUTTON_CAR -> Emergency.Doors.Opening1.Button_detection1.BUTTON_UP
          (junction 92956) -> (junction 92958)
          (junction 92958) -> (junction 92957)
          (junction 92957) -> (junction 92960)
          Emergency.Doors.Opening1.Button_detection1.GoTo_PositionControl -> (junction 92959)
          (junction 92960) -> (junction 92961) [order 1] : [FLAG==1]
          (junction 92961) -> Emergency.Doors.Opening1.Button_detection1.GoTo_PositionControl [order 1] : [PUSHED]
          (junction 92959) -> (junction 92963)
          (junction 92960) -> (junction 92971) [order 2]
          (junction 92961) -> (junction 92962) [order 2]
          (junction 92963) -> (junction 92962)
          (junction 92962) -> (junction 92965)
          Emergency.Doors.Opening1.Button_detection1.Emergency -> (junction 92964)
          (junction 92965) -> Emergency.Doors.Opening1.Button_detection1.Timer_EME [order 1] : [STOP]
              | {IN_LL=false; ET_LL=0;FLAG=1;}
          Emergency.Doors.Opening1.Button_detection1.Timer_EME -> (junction 92966)
          (junction 92966) -> Emergency.Doors.Opening1.Button_detection1.Emergency [order 1] : [Q_EME]
          (junction 92964) -> (junction 92968)
          (junction 92965) -> Emergency.Doors.Opening1.Button_detection1.Not_Emergency [order 2]
          (junction 92966) -> (junction 92967) [order 2]
          (junction 92968) -> (junction 92967)
          (junction 92967) -> (junction 92970)
          Emergency.Doors.Opening1.Button_detection1.Not_Emergency -> (junction 92970)
          Emergency.Doors.Opening1.Button_detection1.SwitchingOFF_LEDs -> (junction 92969)
          (junction 92970) -> Emergency.Doors.Opening1.Button_detection1.SwitchingOFF_LEDs [order 1] : [FLAG_STOP && FLAG==2]
          (junction 92969) -> (junction 92973)
          (junction 92970) -> (junction 92972) [order 2]
          (junction 92972) -> (junction 92971)
          (junction 92973) -> (junction 92972)
        state Opening1
          en:AP1=true;
        state Reset
          state Reset_0
            en:
            LPS0=false;
            BUTTON_CAR(1)=false;
            BUTTON_UP(1)=false;
          state Reset_1
            en:
            LPS1=false;
            LPD1=false;
            BUTTON_CAR(2)=false;
            BUTTON_UP(2)=false;
            BUTTON_DOWN(2)=false;
          state Reset_2
            en:
            LPS2=false;
            LPD2=false;
            BUTTON_CAR(3)=false;
            BUTTON_UP(3)=false;
            BUTTON_DOWN(3)=false;
          state Reset_3
            en:
            LPD3=false;
            BUTTON_CAR(4)=false;
            BUTTON_DOWN(4)=false;
          (default) -> (junction 93367)
          (junction 93367) -> Emergency.Doors.Opening1.Reset.Reset_0 [order 1] : [FLOOR==0]
          Emergency.Doors.Opening1.Reset.Reset_0 -> (junction 93368)
          (junction 93367) -> (junction 93369) [order 2]
          (junction 93368) -> (junction 93370)
          (junction 93369) -> Emergency.Doors.Opening1.Reset.Reset_1 [order 1] : [FLOOR==1]
          Emergency.Doors.Opening1.Reset.Reset_1 -> (junction 93370)
          (junction 93369) -> (junction 93371) [order 2]
          (junction 93370) -> (junction 93372)
          (junction 93371) -> Emergency.Doors.Opening1.Reset.Reset_2 [order 1] : [FLOOR==2]
          Emergency.Doors.Opening1.Reset.Reset_2 -> (junction 93372)
          (junction 93371) -> (junction 93373) [order 2]
          (junction 93372) -> (junction 93374)
          (junction 93373) -> Emergency.Doors.Opening1.Reset.Reset_3 [order 1] : [FLOOR==3]
          Emergency.Doors.Opening1.Reset.Reset_3 -> (junction 93374)
          (junction 93373) -> (junction 93375) [order 2]
          (junction 93374) -> (junction 93376)
          (junction 93376) -> (junction 93375)
        state Stop_Opening1
          en: AP1=false;
          FLAG_OD=true;
          IN_cl=false;
          ET_cl=0;
        (junction 92364) -> (junction 92365)
        (junction 92365) -> (junction 92366) [order 1] : [not(OBS) ]
        (junction 92368) -> Emergency.Doors.Opening1.Opening [order 1] : [not(PA1)]
        (junction 92366) -> (junction 92367) [order 2]
        (junction 92367) -> Emergency.Doors.Opening1.Timer_open
        Emergency.Doors.Opening1.Timer_open -> (junction 92368)
        (default) -> Emergency.Doors.Opening1.People_IN
        (junction 92365) -> (junction 92369) [order 2]
        (junction 92366) -> Emergency.Doors.Opening1.Button_detection [order 1] : [not(FLAG==4)]
        (junction 92371) -> (junction 92367)
        (junction 92373) -> (junction 92364)
        (junction 92368) -> Emergency.Doors.Opening1.Stop_Opening [order 2]
        Emergency.Doors.Opening1.People_IN -> Emergency.Doors.Opening1.People_OUT
        Emergency.Doors.Opening1.Opening -> (junction 92378)
        (junction 92369) -> (junction 92370) [order 2]
        (junction 92369) -> Emergency.Doors.Opening1.Button_detection1 [order 1] : [not(FLAG==4)]
        (junction 92370) -> (junction 92375)
        Emergency.Doors.Opening1.Button_detection -> (junction 92371)
        Emergency.Doors.Opening1.People_OUT -> (junction 92372)
        Emergency.Doors.Opening1.Button_detection1 -> (junction 92374)
        (junction 92375) -> (junction 92374)
        (junction 92372) -> (junction 92373) [order 2]
        (junction 92372) -> Emergency.Doors.Opening1.Reset [order 1] : [not(FLAG==4)]
        (junction 92374) -> (junction 92376)
        (junction 92382) -> (junction 92373)
        Emergency.Doors.Opening1.Stop_Opening -> (junction 92377)
        (junction 92376) -> Emergency.Doors.Opening1.Opening1 [order 1] : [not(PA1)]
        (junction 92376) -> Emergency.Doors.Opening1.Stop_Opening1 [order 2]
        (junction 92378) -> (junction 92377)
        (junction 92377) -> (junction 92380)
        Emergency.Doors.Opening1.Opening1 -> (junction 92379)
        Emergency.Doors.Opening1.Reset -> (junction 92381)
        Emergency.Doors.Opening1.Stop_Opening1 -> (junction 92379)
        (junction 92379) -> (junction 92380)
        (junction 92381) -> (junction 92382)
      state FLOOR_2
        en: CP2=false;
      state Opening2
        state Opening
          en:AP2=Q_op;
        state People_IN
          state Check_People_IN
            en:
            COUNTER_IN=false;
          state People_KID_IN
            en:
            WEIGHT=WEIGHT+30;
            KIDS=KIDS+1;
          state People_WOMAN_IN
            en:
            WEIGHT=WEIGHT+55;
            WOMEN=WOMEN+1;
          state People_MAN_IN
            en:
            WEIGHT=WEIGHT+75;
            MEN=MEN+1;
          state People_FATGUY_IN
            en:
            WEIGHT=WEIGHT+100;
            FATGUYS=FATGUYS+1;
          state Re_Ready_IN
            en:
            COUNTER_IN=true;
          (default) -> (junction 93457)
          (junction 93457) -> Emergency.Doors.Opening2.People_IN.Check_People_IN [order 1] : [COUNTER_IN]
          Emergency.Doors.Opening2.People_IN.Check_People_IN -> (junction 93458)
          (junction 93458) -> Emergency.Doors.Opening2.People_IN.People_KID_IN [order 1] : [KID_IN]
          Emergency.Doors.Opening2.People_IN.People_KID_IN -> (junction 93459)
          (junction 93457) -> (junction 93466) [order 2]
          (junction 93458) -> (junction 93460) [order 2]
          (junction 93459) -> (junction 93461)
          (junction 93460) -> Emergency.Doors.Opening2.People_IN.People_WOMAN_IN [order 1] : [WOMAN_IN]
          Emergency.Doors.Opening2.People_IN.People_WOMAN_IN -> (junction 93461)
          (junction 93460) -> (junction 93462) [order 2]
          (junction 93461) -> (junction 93463)
          (junction 93462) -> Emergency.Doors.Opening2.People_IN.People_MAN_IN [order 1] : [MAN_IN]
          Emergency.Doors.Opening2.People_IN.People_MAN_IN -> (junction 93463)
          (junction 93462) -> (junction 93464) [order 2]
          (junction 93463) -> (junction 93465)
          (junction 93464) -> Emergency.Doors.Opening2.People_IN.People_FATGUY_IN [order 1] : [FATGUY_IN]
          Emergency.Doors.Opening2.People_IN.People_FATGUY_IN -> (junction 93465)
          (junction 93464) -> (junction 93467) [order 2]
          (junction 93465) -> (junction 93468)
          (junction 93467) -> (junction 93466)
          (junction 93468) -> (junction 93467)
          (junction 93466) -> (junction 93469)
          (junction 93469) -> Emergency.Doors.Opening2.People_IN.Re_Ready_IN [order 1] : [not(KID_IN|| WOMAN_IN || MAN_IN || FATGUY_IN)]
          (junction 93469) -> (junction 93470) [order 2]
          Emergency.Doors.Opening2.People_IN.Re_Ready_IN -> (junction 93471)
          (junction 93471) -> (junction 93470)
        state Timer_open
          state Set_tmr
            en: Q_op=true;
          state Set
            en:PT_op=2;
            IN_op=true;
          state Counting
            en:ET_op = ET_op + 1;
            Q_op=false;
          (junction 93506) -> Emergency.Doors.Opening2.Timer_open.Set_tmr [order 1] : [ET_op==PT_op]
          Emergency.Doors.Opening2.Timer_open.Set_tmr -> (junction 93507)
          (default) -> Emergency.Doors.Opening2.Timer_open.Set
          Emergency.Doors.Opening2.Timer_open.Counting -> (junction 93506)
          (junction 93506) -> (junction 93507) [order 2]
          Emergency.Doors.Opening2.Timer_open.Set -> (junction 93508)
          (junction 93508) -> Emergency.Doors.Opening2.Timer_open.Counting [order 1] : [ET_op<PT_op]
          (junction 93508) -> (junction 93507) [order 2]
        state Stop_Opening
          en:AP2=false;
          FLAG_OD=true;
          OBS=true;
          IN_op=false;
          ET_op=0;
        state People_OUT
          state Check_People_OUT
            en:
            COUNTER_OUT=false;
          state People_KID_OUT
            en:
            WEIGHT=WEIGHT-30;
            KIDS=KIDS-1;
          state People_WOMAN_OUT
            en:
            WEIGHT=WEIGHT-55;
            WOMEN=WOMEN-1;
          state People_MAN_OUT
            en:
            WEIGHT=WEIGHT-75;
            MEN=MEN-1;
          state People_FATGUY_OUT
            en:
            WEIGHT=WEIGHT-100;
            FATGUYS=FATGUYS-1;
          state Re_Ready_OUT
            en:
            COUNTER_OUT=true;
          (default) -> (junction 93522)
          (junction 93522) -> Emergency.Doors.Opening2.People_OUT.Check_People_OUT [order 1] : [COUNTER_OUT]
          Emergency.Doors.Opening2.People_OUT.Check_People_OUT -> (junction 93523)
          (junction 93523) -> Emergency.Doors.Opening2.People_OUT.People_KID_OUT [order 1] : [KID_OUT && KIDS>0 ]
          Emergency.Doors.Opening2.People_OUT.People_KID_OUT -> (junction 93524)
          (junction 93522) -> (junction 93531) [order 2]
          (junction 93523) -> (junction 93525) [order 2]
          (junction 93524) -> (junction 93526)
          (junction 93525) -> Emergency.Doors.Opening2.People_OUT.People_WOMAN_OUT [order 1] : [WOMAN_OUT && WOMEN>0]
          Emergency.Doors.Opening2.People_OUT.People_WOMAN_OUT -> (junction 93526)
          (junction 93526) -> (junction 93528)
          (junction 93525) -> (junction 93527) [order 2]
          (junction 93527) -> Emergency.Doors.Opening2.People_OUT.People_MAN_OUT [order 1] : [MAN_OUT && MEN>0]
          Emergency.Doors.Opening2.People_OUT.People_MAN_OUT -> (junction 93528)
          (junction 93527) -> (junction 93529) [order 2]
          (junction 93528) -> (junction 93530)
          (junction 93529) -> Emergency.Doors.Opening2.People_OUT.People_FATGUY_OUT [order 1] : [FATGUY_OUT && FATGUYS>0]
          Emergency.Doors.Opening2.People_OUT.People_FATGUY_OUT -> (junction 93530)
          (junction 93529) -> (junction 93532) [order 2]
          (junction 93530) -> (junction 93533)
          (junction 93532) -> (junction 93531)
          (junction 93533) -> (junction 93532)
          (junction 93531) -> (junction 93534)
          (junction 93534) -> Emergency.Doors.Opening2.People_OUT.Re_Ready_OUT [order 1] : [not(KID_OUT || WOMAN_OUT || MAN_OUT || FATGUY_OUT)]
          (junction 93534) -> (junction 93535) [order 2]
          Emergency.Doors.Opening2.People_OUT.Re_Ready_OUT -> (junction 93536)
          (junction 93536) -> (junction 93535)
        state Button_detection
          state Save_energy
            en:
            LL=not(Q_LL);
          state Timer_LL
            state Set_tmr
              en:
              Q_LL=true;
            state Counting
              en:
              ET_LL= ET_LL + 1;
              Q_LL=false;
            state Set
              en:
              IN_LL=true;
              PT_LL=10;
            (junction 93639) -> Emergency.Doors.Opening2.Button_detection.Timer_LL.Set_tmr [order 1] : [ET_LL==PT_LL]
            Emergency.Doors.Opening2.Button_detection.Timer_LL.Set_tmr -> (junction 93640)
            Emergency.Doors.Opening2.Button_detection.Timer_LL.Counting -> (junction 93639)
            (junction 93639) -> (junction 93640) [order 2]
            (default) -> Emergency.Doors.Opening2.Button_detection.Timer_LL.Set
            Emergency.Doors.Opening2.Button_detection.Timer_LL.Set -> (junction 93641)
            (junction 93641) -> Emergency.Doors.Opening2.Button_detection.Timer_LL.Counting [order 1] : [ET_LL<PT_LL]
            (junction 93641) -> (junction 93640) [order 2]
          state BUTTON_DOWN
            state Button_DOWN_1
              en:
              BUTTON_DOWN(2)=true;
              BUT_TEMP=1;
              LPD1=true;
              PUSHED=true;
              UPDATE=false;
              IN_LL=false; ET_LL=0;
            state First_but_1
              en:
              BUT_1=BUT_TEMP;
              FIRST_BUT=false;
            state Button_DOWN_2
              en:
              BUTTON_DOWN(3)=true;
              BUT_TEMP=2;
              LPD2=true;
              PUSHED=true;
              UPDATE=false;
              IN_LL=false; ET_LL=0;
            state First_but_2
              en:
              BUT_1=BUT_TEMP;
              FIRST_BUT=false;
            state Button_DOWN_3
              en:
              BUTTON_DOWN(4)=true;
              BUT_TEMP=3;
              LPD3=true;
              PUSHED=true;
              UPDATE=false;
              IN_LL=false; ET_LL=0;
            state First_but_3
              en:
              BUT_1=BUT_TEMP;
              FIRST_BUT=false;
            (default) -> (junction 93654)
            (junction 93654) -> Emergency.Doors.Opening2.Button_detection.BUTTON_DOWN.Button_DOWN_1 [order 1] : [PD1]
            Emergency.Doors.Opening2.Button_detection.BUTTON_DOWN.Button_DOWN_1 -> (junction 93655)
            (junction 93655) -> Emergency.Doors.Opening2.Button_detection.BUTTON_DOWN.First_but_1 [order 1] : [FIRST_BUT && not(RPC1)]
            Emergency.Doors.Opening2.Button_detection.BUTTON_DOWN.First_but_1 -> (junction 93656)
            (junction 93654) -> (junction 93657) [order 2]
            (junction 93655) -> (junction 93658) [order 2]
            (junction 93656) -> (junction 93659)
            (junction 93658) -> (junction 93657)
            (junction 93659) -> (junction 93658)
            (junction 93657) -> (junction 93660)
            (junction 93660) -> Emergency.Doors.Opening2.Button_detection.BUTTON_DOWN.Button_DOWN_2 [order 1] : [PD2]
            Emergency.Doors.Opening2.Button_detection.BUTTON_DOWN.Button_DOWN_2 -> (junction 93661)
            (junction 93661) -> Emergency.Doors.Opening2.Button_detection.BUTTON_DOWN.First_but_2 [order 1] : [FIRST_BUT && not(RPC2)]
            Emergency.Doors.Opening2.Button_detection.BUTTON_DOWN.First_but_2 -> (junction 93662)
            (junction 93660) -> (junction 93663) [order 2]
            (junction 93661) -> (junction 93664) [order 2]
            (junction 93662) -> (junction 93665)
            (junction 93664) -> (junction 93663)
            (junction 93665) -> (junction 93664)
            (junction 93663) -> (junction 93666)
            (junction 93666) -> Emergency.Doors.Opening2.Button_detection.BUTTON_DOWN.Button_DOWN_3 [order 1] : [PD3]
            Emergency.Doors.Opening2.Button_detection.BUTTON_DOWN.Button_DOWN_3 -> (junction 93667)
            (junction 93667) -> Emergency.Doors.Opening2.Button_detection.BUTTON_DOWN.First_but_3 [order 1] : [FIRST_BUT && not(RPC3)]
            Emergency.Doors.Opening2.Button_detection.BUTTON_DOWN.First_but_3 -> (junction 93668)
            (junction 93666) -> (junction 93669) [order 2]
            (junction 93667) -> (junction 93670) [order 2]
            (junction 93668) -> (junction 93671)
            (junction 93670) -> (junction 93669)
            (junction 93671) -> (junction 93670)
          state BUTTON_CAR
            state Button_CAR_0
              en:
              BUTTON_CAR(1)=true;
              BUT_TEMP=0;
              LPC0=true;
              PUSHED=true;
              UPDATE=false;
              IN_LL=false; ET_LL=0;
            state First_but_0
              en:
              BUT_1=BUT_TEMP;
              FIRST_BUT=false;
            state Button_CAR_1
              en:
              BUTTON_CAR(2)=true;
              BUT_TEMP=1;
              LPC1=true;
              PUSHED=true;
              UPDATE=false;
              IN_LL=false; ET_LL=0;
            state First_but_1
              en:
              BUT_1=BUT_TEMP;
              FIRST_BUT=false;
            state Button_CAR_2
              en:
              BUTTON_CAR(3)=true;
              BUT_TEMP=2;
              LPC2=true;
              PUSHED=true;
              UPDATE=false;
              IN_LL=false; ET_LL=0;
            state First_but_2
              en:
              BUT_1=BUT_TEMP;
              FIRST_BUT=false;
            state Button_CAR_3
              en:
              BUTTON_CAR(4)=true;
              BUT_TEMP=3;
              LPC3=true;
              PUSHED=true;
              UPDATE=false;
              IN_LL=false; ET_LL=0;
            state First_but_3
              en:
              BUT_1=BUT_TEMP;
              FIRST_BUT=false;
            (default) -> (junction 93709)
            (junction 93709) -> Emergency.Doors.Opening2.Button_detection.BUTTON_CAR.Button_CAR_0 [order 1] : [P0]
            Emergency.Doors.Opening2.Button_detection.BUTTON_CAR.Button_CAR_0 -> (junction 93710)
            (junction 93710) -> Emergency.Doors.Opening2.Button_detection.BUTTON_CAR.First_but_0 [order 1] : [FIRST_BUT && not(RPC0)]
            Emergency.Doors.Opening2.Button_detection.BUTTON_CAR.First_but_0 -> (junction 93711)
            (junction 93709) -> (junction 93712) [order 2]
            (junction 93710) -> (junction 93713) [order 2]
            (junction 93711) -> (junction 93714)
            (junction 93713) -> (junction 93712)
            (junction 93714) -> (junction 93713)
            (junction 93712) -> (junction 93717)
            Emergency.Doors.Opening2.Button_detection.BUTTON_CAR.Button_CAR_1 -> (junction 93715)
            (junction 93715) -> Emergency.Doors.Opening2.Button_detection.BUTTON_CAR.First_but_1 [order 1] : [FIRST_BUT && not(RPC1)]
            Emergency.Doors.Opening2.Button_detection.BUTTON_CAR.First_but_1 -> (junction 93716)
            (junction 93715) -> (junction 93719) [order 2]
            (junction 93716) -> (junction 93720)
            (junction 93717) -> Emergency.Doors.Opening2.Button_detection.BUTTON_CAR.Button_CAR_1 [order 1] : [P1]
            (junction 93717) -> (junction 93718) [order 2]
            (junction 93719) -> (junction 93718)
            (junction 93720) -> (junction 93719)
            (junction 93718) -> (junction 93721)
            (junction 93721) -> Emergency.Doors.Opening2.Button_detection.BUTTON_CAR.Button_CAR_2 [order 1] : [P2]
            Emergency.Doors.Opening2.Button_detection.BUTTON_CAR.Button_CAR_2 -> (junction 93722)
            (junction 93722) -> Emergency.Doors.Opening2.Button_detection.BUTTON_CAR.First_but_2 [order 1] : [FIRST_BUT && not(RPC2)]
            Emergency.Doors.Opening2.Button_detection.BUTTON_CAR.First_but_2 -> (junction 93723)
            (junction 93721) -> (junction 93724) [order 2]
            (junction 93722) -> (junction 93725) [order 2]
            (junction 93723) -> (junction 93726)
            (junction 93725) -> (junction 93724)
            (junction 93726) -> (junction 93725)
            (junction 93724) -> (junction 93727)
            (junction 93727) -> Emergency.Doors.Opening2.Button_detection.BUTTON_CAR.Button_CAR_3 [order 1] : [P3]
            Emergency.Doors.Opening2.Button_detection.BUTTON_CAR.Button_CAR_3 -> (junction 93728)
            (junction 93728) -> Emergency.Doors.Opening2.Button_detection.BUTTON_CAR.First_but_3 [order 1] : [FIRST_BUT && not(RPC3)]
            Emergency.Doors.Opening2.Button_detection.BUTTON_CAR.First_but_3 -> (junction 93729)
            (junction 93727) -> (junction 93730) [order 2]
            (junction 93728) -> (junction 93731) [order 2]
            (junction 93729) -> (junction 93732)
            (junction 93731) -> (junction 93730)
            (junction 93732) -> (junction 93731)
          state BUTTON_UP
            state Button_UP_0
              en:
              BUTTON_UP(1)=true;
              BUT_TEMP=0;
              LPS0=true;
              PUSHED=true;
              UPDATE=false;
              IN_LL=false; ET_LL=0;
            state First_but_0
              en:
              BUT_1=BUT_TEMP;
              FIRST_BUT=false;
            state Button_UP_1
              en:
              BUTTON_UP(2)=true;
              BUT_TEMP=1;
              LPS1=true;
              PUSHED=true;
              UPDATE=false;
              IN_LL=false; ET_LL=0;
            state First_but_1
              en:
              BUT_1=BUT_TEMP;
              FIRST_BUT=false;
            state Button_UP_2
              en:
              BUTTON_UP(3)=true;
              BUT_TEMP=2;
              LPS2=true;
              PUSHED=true;
              UPDATE=false;
              IN_LL=false; ET_LL=0;
            state First_but_2
              en:
              BUT_1=BUT_TEMP;
              FIRST_BUT=false;
            (junction 93782) -> Emergency.Doors.Opening2.Button_detection.BUTTON_UP.Button_UP_0 [order 1] : [PS0]
            Emergency.Doors.Opening2.Button_detection.BUTTON_UP.Button_UP_0 -> (junction 93783)
            (junction 93783) -> Emergency.Doors.Opening2.Button_detection.BUTTON_UP.First_but_0 [order 1] : [FIRST_BUT && not(RPC0)]
            Emergency.Doors.Opening2.Button_detection.BUTTON_UP.First_but_0 -> (junction 93784)
            (default) -> (junction 93782)
            (junction 93782) -> (junction 93787) [order 2]
            (junction 93783) -> (junction 93785) [order 2]
            (junction 93784) -> (junction 93786)
            (junction 93786) -> (junction 93785)
            (junction 93785) -> (junction 93787)
            (junction 93787) -> (junction 93788)
            (junction 93788) -> Emergency.Doors.Opening2.Button_detection.BUTTON_UP.Button_UP_1 [order 1] : [PS1]
            Emergency.Doors.Opening2.Button_detection.BUTTON_UP.Button_UP_1 -> (junction 93789)
            (junction 93789) -> Emergency.Doors.Opening2.Button_detection.BUTTON_UP.First_but_1 [order 1] : [FIRST_BUT && not(RPC1)]
            Emergency.Doors.Opening2.Button_detection.BUTTON_UP.First_but_1 -> (junction 93790)
            (junction 93788) -> (junction 93791) [order 2]
            (junction 93789) -> (junction 93792) [order 2]
            (junction 93790) -> (junction 93793)
            (junction 93792) -> (junction 93791)
            (junction 93793) -> (junction 93792)
            (junction 93791) -> (junction 93795)
            Emergency.Doors.Opening2.Button_detection.BUTTON_UP.First_but_2 -> (junction 93794)
            (junction 93794) -> (junction 93799)
            (junction 93795) -> Emergency.Doors.Opening2.Button_detection.BUTTON_UP.Button_UP_2 [order 1] : [PS2]
            Emergency.Doors.Opening2.Button_detection.BUTTON_UP.Button_UP_2 -> (junction 93796)
            (junction 93796) -> Emergency.Doors.Opening2.Button_detection.BUTTON_UP.First_but_2 [order 1] : [FIRST_BUT && not(RPC2)]
            (junction 93795) -> (junction 93797) [order 2]
            (junction 93796) -> (junction 93798) [order 2]
            (junction 93798) -> (junction 93797)
            (junction 93799) -> (junction 93798)
          state Max_Min_assignment
            state Min_but
              en:
              BUTTON=MIN_BUT;
            state Max_but
              en:
              BUTTON=MAX_BUT;
            state First_but
              en:
              BUTTON=BUT_1;
            state Max_but1
              en:
              MAX_BUT=2;
            state Max_but2
              en:
              MAX_BUT=1;
            state Max_but3
              en:
              MAX_BUT=0;
            state Min_but1
              en:
              MIN_BUT=1;
            state Min_but2
              en:
              MIN_BUT=2;
            state Min_but3
              en:
              MIN_BUT=3;
            state MAX
              en:
              MAX_BUT=BUT_TEMP;
            state MIN
              en:
              MIN_BUT=BUT_TEMP;
            state Updating_button_0
              en:
              BUTTON=MAX_BUT;
            state Updating_button_1
              en:
              BUTTON=MIN_BUT;
            (junction 93837) -> Emergency.Doors.Opening2.Button_detection.Max_Min_assignment.Min_but [order 1] : [(MAX_BUT-FLOOR)>(FLOOR-MIN_BUT)]
            Emergency.Doors.Opening2.Button_detection.Max_Min_assignment.Min_but -> (junction 93838)
            (junction 93839) -> (junction 93837) [order 1] : [not(FLAG_STOP) && MOTION==2 && FLAG==3]
            (default) -> (junction 93839)
            (junction 93837) -> (junction 93840) [order 2]
            (junction 93838) -> (junction 93841)
            (junction 93839) -> (junction 93842) [order 2]
            (junction 93840) -> Emergency.Doors.Opening2.Button_detection.Max_Min_assignment.Max_but [order 1] : [(MAX_BUT-FLOOR)<(FLOOR-MIN_BUT)]
            Emergency.Doors.Opening2.Button_detection.Max_Min_assignment.Max_but -> (junction 93841)
            (junction 93840) -> Emergency.Doors.Opening2.Button_detection.Max_Min_assignment.First_but [order 2]
            (junction 93841) -> (junction 93844)
            Emergency.Doors.Opening2.Button_detection.Max_Min_assignment.First_but -> (junction 93843)
            (junction 93843) -> (junction 93842)
            (junction 93844) -> (junction 93843)
            (junction 93842) -> (junction 93845)
            (junction 93846) -> (junction 93847) [order 1] : [MOTION==0]
                | {MOTION=1;
                | UPDATE=true;}
            (junction 93847) -> Emergency.Doors.Opening2.Button_detection.Max_Min_assignment.Max_but1 [order 1] : [BUTTON_UP(2)]
            Emergency.Doors.Opening2.Button_detection.Max_Min_assignment.Max_but1 -> (junction 93848)
            (junction 93845) -> (junction 93846) [order 1] : [BUTTON==FLOOR && EXTEND]
                | {EXTEND=false;}
            (junction 93845) -> (junction 93859) [order 2]
            (junction 93846) -> (junction 93851) [order 2]
            (junction 93847) -> (junction 93849) [order 2]
            (junction 93848) -> (junction 93850)
            (junction 93849) -> Emergency.Doors.Opening2.Button_detection.Max_Min_assignment.Max_but2 [order 1] : [BUTTON_UP(1)]
            Emergency.Doors.Opening2.Button_detection.Max_Min_assignment.Max_but2 -> (junction 93850)
            (junction 93849) -> Emergency.Doors.Opening2.Button_detection.Max_Min_assignment.Max_but3 [order 2]
            (junction 93850) -> (junction 93853)
            Emergency.Doors.Opening2.Button_detection.Max_Min_assignment.Max_but3 -> (junction 93852)
            (junction 93852) -> (junction 93851)
            (junction 93853) -> (junction 93852)
            (junction 93851) -> (junction 93854)
            (junction 93854) -> (junction 93855) [order 1] : [MOTION==1]
                | {MOTION=0;
                | UPDATE=true;}
            (junction 93855) -> Emergency.Doors.Opening2.Button_detection.Max_Min_assignment.Min_but1 [order 1] : [BUTTON_DOWN(1)]
            Emergency.Doors.Opening2.Button_detection.Max_Min_assignment.Min_but1 -> (junction 93856)
            (junction 93854) -> (junction 93860) [order 2]
            (junction 93855) -> (junction 93857) [order 2]
            (junction 93856) -> (junction 93858)
            (junction 93857) -> Emergency.Doors.Opening2.Button_detection.Max_Min_assignment.Min_but2 [order 1] : [BUTTON_DOWN(2)]
            Emergency.Doors.Opening2.Button_detection.Max_Min_assignment.Min_but2 -> (junction 93858)
            (junction 93857) -> Emergency.Doors.Opening2.Button_detection.Max_Min_assignment.Min_but3 [order 2]
            (junction 93858) -> (junction 93862)
            Emergency.Doors.Opening2.Button_detection.Max_Min_assignment.Min_but3 -> (junction 93861)
            (junction 93860) -> (junction 93859)
            (junction 93861) -> (junction 93860)
            (junction 93862) -> (junction 93861)
            (junction 93859) -> (junction 93864)
            Emergency.Doors.Opening2.Button_detection.Max_Min_assignment.MAX -> (junction 93863)
            (junction 93864) -> (junction 93865) [order 1] : [PUSHED]
            (junction 93865) -> (junction 93866) [order 1] : [not(BUT_TEMP==FLOOR) || not(MOTION==2)]
            (junction 93866) -> Emergency.Doors.Opening2.Button_detection.Max_Min_assignment.MAX [order 1] : [MAX_BUT<BUT_TEMP && not(UPDATE)]
            (junction 93863) -> (junction 93868)
            (junction 93864) -> (junction 93878) [order 2]
            (junction 93865) -> (junction 93871) [order 2]
            (junction 93866) -> (junction 93867) [order 2]
            (junction 93868) -> (junction 93867)
            (junction 93867) -> (junction 93869)
            (junction 93869) -> Emergency.Doors.Opening2.Button_detection.Max_Min_assignment.MIN [order 1] : [MIN_BUT>BUT_TEMP && not(UPDATE)]
            Emergency.Doors.Opening2.Button_detection.Max_Min_assignment.MIN -> (junction 93870)
            (junction 93869) -> (junction 93872) [order 2]
            (junction 93870) -> (junction 93873)
            (junction 93872) -> (junction 93871)
            (junction 93873) -> (junction 93872)
            (junction 93871) -> (junction 93874)
            (junction 93874) -> Emergency.Doors.Opening2.Button_detection.Max_Min_assignment.Updating_button_0 [order 1] : [MOTION==0]
            Emergency.Doors.Opening2.Button_detection.Max_Min_assignment.Updating_button_0 -> (junction 93875)
            (junction 93874) -> (junction 93876) [order 2]
            (junction 93875) -> (junction 93877)
            (junction 93876) -> Emergency.Doors.Opening2.Button_detection.Max_Min_assignment.Updating_button_1 [order 1] : [MOTION==1]
            Emergency.Doors.Opening2.Button_detection.Max_Min_assignment.Updating_button_1 -> (junction 93877)
            (junction 93876) -> (junction 93879) [order 2]
            (junction 93877) -> (junction 93880)
            (junction 93879) -> (junction 93878)
            (junction 93880) -> (junction 93879)
          state GoTo_PositionControl
            en:
            BUTTON=BUT_TEMP;
            FLAG=2;
          state Emergency
            en:
            FLAG_EMG=true;
            FLAG=4;
          state Timer_EME
            state Set_tmr
              en:
              Q_EME=true;
            state Counting
              en:
              ET_EME= ET_EME + 1;
              Q_EME=false;
            state Set
              en:
              IN_EME=true;
              PT_EME=3;
            (junction 93970) -> Emergency.Doors.Opening2.Button_detection.Timer_EME.Set_tmr [order 1] : [ET_EME==PT_EME]
            Emergency.Doors.Opening2.Button_detection.Timer_EME.Set_tmr -> (junction 93971)
            Emergency.Doors.Opening2.Button_detection.Timer_EME.Counting -> (junction 93970)
            (junction 93970) -> (junction 93971) [order 2]
            (default) -> Emergency.Doors.Opening2.Button_detection.Timer_EME.Set
            Emergency.Doors.Opening2.Button_detection.Timer_EME.Set -> (junction 93972)
            (junction 93972) -> Emergency.Doors.Opening2.Button_detection.Timer_EME.Counting [order 1] : [ET_EME<PT_EME]
            (junction 93972) -> (junction 93971) [order 2]
          state Not_Emergency
            en:
            IN_EME=false;
            ET_EME=0;
          state SwitchingOFF_LEDs
            en:
            LPD3=false;
            LPD2=false;
            LPS2=false;
            LPD1=false;
            LPS1=false;
            LPS0=false;
          (default) -> (junction 93571)
          (junction 93571) -> (junction 93572) [order 1] : [FLAG==1 && not(PUSHED)]
              | {BUTTON=FLOOR;
              | BUT_TEMP=BUTTON;
              | BUT_1=FLOOR;}
          (junction 93572) -> Emergency.Doors.Opening2.Button_detection.Timer_LL [order 1] : [not(FLAG_STOP)]
          Emergency.Doors.Opening2.Button_detection.Timer_LL -> Emergency.Doors.Opening2.Button_detection.Save_energy
          Emergency.Doors.Opening2.Button_detection.Save_energy -> (junction 93573)
          (junction 93571) -> (junction 93574) [order 2]
          (junction 93572) -> (junction 93575) [order 2]
          (junction 93573) -> (junction 93576)
          (junction 93575) -> (junction 93574)
          (junction 93576) -> (junction 93575)
          (junction 93574) -> Emergency.Doors.Opening2.Button_detection.BUTTON_CAR
          Emergency.Doors.Opening2.Button_detection.BUTTON_UP -> Emergency.Doors.Opening2.Button_detection.BUTTON_DOWN
          Emergency.Doors.Opening2.Button_detection.BUTTON_DOWN -> Emergency.Doors.Opening2.Button_detection.Max_Min_assignment
          Emergency.Doors.Opening2.Button_detection.Max_Min_assignment -> (junction 93577)
          Emergency.Doors.Opening2.Button_detection.BUTTON_CAR -> Emergency.Doors.Opening2.Button_detection.BUTTON_UP
          (junction 93577) -> (junction 93579)
          (junction 93579) -> (junction 93578)
          (junction 93578) -> (junction 93580)
          (junction 93580) -> (junction 93581) [order 1] : [FLAG==1]
          (junction 93581) -> Emergency.Doors.Opening2.Button_detection.GoTo_PositionControl [order 1] : [PUSHED]
          Emergency.Doors.Opening2.Button_detection.GoTo_PositionControl -> (junction 93582)
          (junction 93580) -> (junction 93592) [order 2]
          (junction 93581) -> (junction 93583) [order 2]
          (junction 93582) -> (junction 93584)
          (junction 93584) -> (junction 93583)
          (junction 93583) -> (junction 93586)
          Emergency.Doors.Opening2.Button_detection.Emergency -> (junction 93585)
          (junction 93586) -> Emergency.Doors.Opening2.Button_detection.Timer_EME [order 1] : [STOP]
              | {IN_LL=false; ET_LL=0;FLAG=1;}
          Emergency.Doors.Opening2.Button_detection.Timer_EME -> (junction 93587)
          (junction 93587) -> Emergency.Doors.Opening2.Button_detection.Emergency [order 1] : [Q_EME]
          (junction 93585) -> (junction 93589)
          (junction 93586) -> Emergency.Doors.Opening2.Button_detection.Not_Emergency [order 2]
          (junction 93587) -> (junction 93588) [order 2]
          (junction 93589) -> (junction 93588)
          (junction 93588) -> (junction 93591)
          Emergency.Doors.Opening2.Button_detection.Not_Emergency -> (junction 93591)
          Emergency.Doors.Opening2.Button_detection.SwitchingOFF_LEDs -> (junction 93590)
          (junction 93591) -> Emergency.Doors.Opening2.Button_detection.SwitchingOFF_LEDs [order 1] : [FLAG_STOP && FLAG==2]
          (junction 93590) -> (junction 93594)
          (junction 93591) -> (junction 93593) [order 2]
          (junction 93593) -> (junction 93592)
          (junction 93594) -> (junction 93593)
        state Button_detection1
          state Save_energy
            en:
            LL=not(Q_LL);
          state Timer_LL
            state Set_tmr
              en:
              Q_LL=true;
            state Counting
              en:
              ET_LL= ET_LL + 1;
              Q_LL=false;
            state Set
              en:
              IN_LL=true;
              PT_LL=10;
            (junction 94055) -> Emergency.Doors.Opening2.Button_detection1.Timer_LL.Set_tmr [order 1] : [ET_LL==PT_LL]
            Emergency.Doors.Opening2.Button_detection1.Timer_LL.Set_tmr -> (junction 94056)
            Emergency.Doors.Opening2.Button_detection1.Timer_LL.Counting -> (junction 94055)
            (junction 94055) -> (junction 94056) [order 2]
            (default) -> Emergency.Doors.Opening2.Button_detection1.Timer_LL.Set
            Emergency.Doors.Opening2.Button_detection1.Timer_LL.Set -> (junction 94057)
            (junction 94057) -> Emergency.Doors.Opening2.Button_detection1.Timer_LL.Counting [order 1] : [ET_LL<PT_LL]
            (junction 94057) -> (junction 94056) [order 2]
          state BUTTON_DOWN
            state Button_DOWN_1
              en:
              BUTTON_DOWN(2)=true;
              BUT_TEMP=1;
              LPD1=true;
              PUSHED=true;
              UPDATE=false;
              IN_LL=false; ET_LL=0;
            state First_but_1
              en:
              BUT_1=BUT_TEMP;
              FIRST_BUT=false;
            state Button_DOWN_2
              en:
              BUTTON_DOWN(3)=true;
              BUT_TEMP=2;
              LPD2=true;
              PUSHED=true;
              UPDATE=false;
              IN_LL=false; ET_LL=0;
            state First_but_2
              en:
              BUT_1=BUT_TEMP;
              FIRST_BUT=false;
            state Button_DOWN_3
              en:
              BUTTON_DOWN(4)=true;
              BUT_TEMP=3;
              LPD3=true;
              PUSHED=true;
              UPDATE=false;
              IN_LL=false; ET_LL=0;
            state First_but_3
              en:
              BUT_1=BUT_TEMP;
              FIRST_BUT=false;
            (default) -> (junction 94070)
            (junction 94070) -> Emergency.Doors.Opening2.Button_detection1.BUTTON_DOWN.Button_DOWN_1 [order 1] : [PD1]
            Emergency.Doors.Opening2.Button_detection1.BUTTON_DOWN.Button_DOWN_1 -> (junction 94071)
            (junction 94071) -> Emergency.Doors.Opening2.Button_detection1.BUTTON_DOWN.First_but_1 [order 1] : [FIRST_BUT && not(RPC1)]
            Emergency.Doors.Opening2.Button_detection1.BUTTON_DOWN.First_but_1 -> (junction 94072)
            (junction 94070) -> (junction 94073) [order 2]
            (junction 94071) -> (junction 94074) [order 2]
            (junction 94072) -> (junction 94075)
            (junction 94074) -> (junction 94073)
            (junction 94075) -> (junction 94074)
            (junction 94073) -> (junction 94076)
            (junction 94076) -> Emergency.Doors.Opening2.Button_detection1.BUTTON_DOWN.Button_DOWN_2 [order 1] : [PD2]
            Emergency.Doors.Opening2.Button_detection1.BUTTON_DOWN.Button_DOWN_2 -> (junction 94077)
            (junction 94077) -> Emergency.Doors.Opening2.Button_detection1.BUTTON_DOWN.First_but_2 [order 1] : [FIRST_BUT && not(RPC2)]
            Emergency.Doors.Opening2.Button_detection1.BUTTON_DOWN.First_but_2 -> (junction 94078)
            (junction 94076) -> (junction 94079) [order 2]
            (junction 94077) -> (junction 94080) [order 2]
            (junction 94078) -> (junction 94081)
            (junction 94080) -> (junction 94079)
            (junction 94081) -> (junction 94080)
            (junction 94079) -> (junction 94082)
            (junction 94082) -> Emergency.Doors.Opening2.Button_detection1.BUTTON_DOWN.Button_DOWN_3 [order 1] : [PD3]
            Emergency.Doors.Opening2.Button_detection1.BUTTON_DOWN.Button_DOWN_3 -> (junction 94083)
            (junction 94083) -> Emergency.Doors.Opening2.Button_detection1.BUTTON_DOWN.First_but_3 [order 1] : [FIRST_BUT && not(RPC3)]
            Emergency.Doors.Opening2.Button_detection1.BUTTON_DOWN.First_but_3 -> (junction 94084)
            (junction 94082) -> (junction 94085) [order 2]
            (junction 94083) -> (junction 94086) [order 2]
            (junction 94084) -> (junction 94087)
            (junction 94086) -> (junction 94085)
            (junction 94087) -> (junction 94086)
          state BUTTON_CAR
            state Button_CAR_0
              en:
              BUTTON_CAR(1)=true;
              BUT_TEMP=0;
              LPC0=true;
              PUSHED=true;
              UPDATE=false;
              IN_LL=false; ET_LL=0;
            state First_but_0
              en:
              BUT_1=BUT_TEMP;
              FIRST_BUT=false;
            state Button_CAR_1
              en:
              BUTTON_CAR(2)=true;
              BUT_TEMP=1;
              LPC1=true;
              PUSHED=true;
              UPDATE=false;
              IN_LL=false; ET_LL=0;
            state First_but_1
              en:
              BUT_1=BUT_TEMP;
              FIRST_BUT=false;
            state Button_CAR_2
              en:
              BUTTON_CAR(3)=true;
              BUT_TEMP=2;
              LPC2=true;
              PUSHED=true;
              UPDATE=false;
              IN_LL=false; ET_LL=0;
            state First_but_2
              en:
              BUT_1=BUT_TEMP;
              FIRST_BUT=false;
            state Button_CAR_3
              en:
              BUTTON_CAR(4)=true;
              BUT_TEMP=3;
              LPC3=true;
              PUSHED=true;
              UPDATE=false;
              IN_LL=false; ET_LL=0;
            state First_but_3
              en:
              BUT_1=BUT_TEMP;
              FIRST_BUT=false;
            (default) -> (junction 94125)
            (junction 94125) -> Emergency.Doors.Opening2.Button_detection1.BUTTON_CAR.Button_CAR_0 [order 1] : [P0]
            Emergency.Doors.Opening2.Button_detection1.BUTTON_CAR.Button_CAR_0 -> (junction 94126)
            (junction 94126) -> Emergency.Doors.Opening2.Button_detection1.BUTTON_CAR.First_but_0 [order 1] : [FIRST_BUT && not(RPC0)]
            Emergency.Doors.Opening2.Button_detection1.BUTTON_CAR.First_but_0 -> (junction 94127)
            (junction 94125) -> (junction 94128) [order 2]
            (junction 94126) -> (junction 94129) [order 2]
            (junction 94127) -> (junction 94130)
            (junction 94129) -> (junction 94128)
            (junction 94130) -> (junction 94129)
            (junction 94128) -> (junction 94133)
            Emergency.Doors.Opening2.Button_detection1.BUTTON_CAR.Button_CAR_1 -> (junction 94131)
            (junction 94131) -> Emergency.Doors.Opening2.Button_detection1.BUTTON_CAR.First_but_1 [order 1] : [FIRST_BUT && not(RPC1)]
            Emergency.Doors.Opening2.Button_detection1.BUTTON_CAR.First_but_1 -> (junction 94132)
            (junction 94131) -> (junction 94135) [order 2]
            (junction 94132) -> (junction 94136)
